simulink model "COMPONENT_MDL_Lag_QUAD_and_PEND_with_Ab"  (R2020b)
(part 12 of 12)

-m_pend.*(-THE_X_D+((Lz_pend.*THE_Psi_pend_D.*cos(THE_Theta_pend).*sin(THE_Psi_pend))./2.0+(Lz_pend.*THE_Theta_pend_D.*cos(THE_Psi_pend).*sin(THE_Theta_pend))./2.0).*(sin(THE_Phi).*sin(THE_Psi)+cos(THE_Phi).*cos(THE_Psi).*sin(THE_Theta))-(Tv_Z_pend+(Lz_pend.*cos(THE_Psi_pend).*cos(THE_Theta_pend))./2.0).*(THE_Phi_D.*cos(THE_Phi).*sin(THE_Psi)+THE_Psi_D.*cos(THE_Psi).*sin(THE_Phi)+THE_Theta_D.*cos(THE_Phi).*cos(THE_Psi).*cos(THE_Theta)-THE_Phi_D.*cos(THE_Psi).*sin(THE_Phi).*sin(THE_Theta)-THE_Psi_D.*cos(THE_Phi).*sin(THE_Psi).*sin(THE_Theta))+(Lz_pend.*(cos(THE_Phi_pend).*sin(THE_Psi_pend)-cos(THE_Psi_pend).*sin(THE_Phi_pend).*sin(THE_Theta_pend)).*(-THE_Phi_D.*cos(THE_Phi).*cos(THE_Psi)+THE_Psi_D.*sin(THE_Phi).*sin(THE_Psi)-THE_Phi_D.*sin(THE_Phi).*sin(THE_Psi).*sin(THE_Theta)+THE_Psi_D.*cos(THE_Phi).*cos(THE_Psi).*sin(THE_Theta)+THE_Theta_D.*cos(THE_Phi).*cos(THE_Theta).*sin(THE_Psi)))./2.0+(Lz_pend.*(cos(THE_Psi).*sin(THE_Phi)-cos(THE_Phi).*sin(THE_Psi).*sin(THE_Theta)).*(-THE_Psi_pend_D.*cos(THE_Phi_pend).*cos(THE_Psi_pend)+THE_Phi_pend_D.*sin(THE_Phi_pend).*sin(THE_Psi_pend)-THE_Psi_pend_D.*sin(THE_Phi_pend).*sin(THE_Psi_pend).*sin(THE_Theta_pend)+THE_Phi_pend_D.*cos(THE_Phi_pend).*cos(THE_Psi_pend).*sin(THE_Theta_pend)+THE_Theta_pend_D.*cos(THE_Psi_pend).*cos(THE_Theta_pend).*sin(THE_Phi_pend)))./2.0-(Lz_pend.*cos(THE_Phi).*cos(THE_Theta).*(THE_Phi_pend_D.*cos(THE_Phi_pend).*sin(THE_Psi_pend)+THE_Psi_pend_D.*cos(THE_Psi_pend).*sin(THE_Phi_pend)+THE_Theta_pend_D.*cos(THE_Phi_pend).*cos(THE_Psi_pend).*cos(THE_Theta_pend)-THE_Phi_pend_D.*cos(THE_Psi_pend).*sin(THE_Phi_pend).*sin(THE_Theta_pend)-THE_Psi_pend_D.*cos(THE_Phi_pend).*sin(THE_Psi_pend).*sin(THE_Theta_pend)))./2.0+(Lz_pend.*THE_Phi_D.*cos(THE_Theta).*sin(THE_Phi).*(sin(THE_Phi_pend).*sin(THE_Psi_pend)+cos(THE_Phi_pend).*cos(THE_Psi_pend).*sin(THE_Theta_pend)))./2.0+(Lz_pend.*THE_Theta_D.*cos(THE_Phi).*sin(THE_Theta).*(sin(THE_Phi_pend).*sin(THE_Psi_pend)+cos(THE_Phi_pend).*cos(THE_Psi_pend).*sin(THE_Theta_pend)))./2.0).*((Lz_pend.*(cos(THE_Phi_pend).*cos(THE_Psi_pend)+sin(THE_Phi_pend).*sin(THE_Psi_pend).*sin(THE_Theta_pend)).*(-THE_Phi_D.*cos(THE_Phi).*cos(THE_Psi)+THE_Psi_D.*sin(THE_Phi).*sin(THE_Psi)-THE_Phi_D.*sin(THE_Phi).*sin(THE_Psi).*sin(THE_Theta)+THE_Psi_D.*cos(THE_Phi).*cos(THE_Psi).*sin(THE_Theta)+THE_Theta_D.*cos(THE_Phi).*cos(THE_Theta).*sin(THE_Psi)))./4.0-(Lz_pend.*(cos(THE_Psi).*sin(THE_Phi)-cos(THE_Phi).*sin(THE_Psi).*sin(THE_Theta)).*(-THE_Phi_pend_D.*cos(THE_Psi_pend).*sin(THE_Phi_pend)-THE_Psi_pend_D.*cos(THE_Phi_pend).*sin(THE_Psi_pend)+THE_Phi_pend_D.*cos(THE_Phi_pend).*sin(THE_Psi_pend).*sin(THE_Theta_pend)+THE_Psi_pend_D.*cos(THE_Psi_pend).*sin(THE_Phi_pend).*sin(THE_Theta_pend)+THE_Theta_pend_D.*cos(THE_Theta_pend).*sin(THE_Phi_pend).*sin(THE_Psi_pend)))./4.0+(Lz_pend.*cos(THE_Theta_pend).*sin(THE_Psi_pend).*(THE_Phi_D.*cos(THE_Phi).*sin(THE_Psi)+THE_Psi_D.*cos(THE_Psi).*sin(THE_Phi)+THE_Theta_D.*cos(THE_Phi).*cos(THE_Psi).*cos(THE_Theta)-THE_Phi_D.*cos(THE_Psi).*sin(THE_Phi).*sin(THE_Theta)-THE_Psi_D.*cos(THE_Phi).*sin(THE_Psi).*sin(THE_Theta)))./4.0+(Lz_pend.*cos(THE_Phi).*cos(THE_Theta).*(-THE_Phi_pend_D.*cos(THE_Phi_pend).*cos(THE_Psi_pend)+THE_Psi_pend_D.*sin(THE_Phi_pend).*sin(THE_Psi_pend)-THE_Phi_pend_D.*sin(THE_Phi_pend).*sin(THE_Psi_pend).*sin(THE_Theta_pend)+THE_Psi_pend_D.*cos(THE_Phi_pend).*cos(THE_Psi_pend).*sin(THE_Theta_pend)+THE_Theta_pend_D.*cos(THE_Phi_pend).*cos(THE_Theta_pend).*sin(THE_Psi_pend)))./4.0+(Lz_pend.*THE_Psi_pend_D.*cos(THE_Psi_pend).*cos(THE_Theta_pend).*(sin(THE_Phi).*sin(THE_Psi)+cos(THE_Phi).*cos(THE_Psi).*sin(THE_Theta)))./4.0+(Lz_pend.*THE_Phi_D.*cos(THE_Theta).*sin(THE_Phi).*(cos(THE_Psi_pend).*sin(THE_Phi_pend)-cos(THE_Phi_pend).*sin(THE_Psi_pend).*sin(THE_Theta_pend)))./4.0+(Lz_pend.*THE_Theta_D.*cos(THE_Phi).*sin(THE_Theta).*(cos(THE_Psi_pend).*sin(THE_Phi_pend)-cos(THE_Phi_pend).*sin(THE_Psi_pend).*sin(THE_Theta_pend)))./4.0-(Lz_pend.*THE_Theta_pend_D.*sin(THE_Psi_pend).*sin(THE_Theta_pend).*(sin(THE_Phi).*sin(THE_Psi)+cos(THE_Phi).*cos(THE_Psi).*sin(THE_Theta)))./4.0)-m_pend.*(THE_X_D.*(-1.0./2.0)+(((Lz_pend.*THE_Psi_pend_D.*cos(THE_Theta_pend).*sin(THE_Psi_pend))./2.0+(Lz_pend.*THE_Theta_pend_D.*cos(THE_Psi_pend).*sin(THE_Theta_pend))./2.0).*(sin(THE_Phi).*sin(THE_Psi)+cos(THE_Phi).*cos(THE_Psi).*sin(THE_Theta)))./2.0-((Tv_Z_pend+(Lz_pend.*cos(THE_Psi_pend).*cos(THE_Theta_pend))./2.0).*(THE_Phi_D.*cos(THE_Phi).*sin(THE_Psi)+THE_Psi_D.*cos(THE_Psi).*sin(THE_Phi)+THE_Theta_D.*cos(THE_Phi).*cos(THE_Psi).*cos(THE_Theta)-THE_Phi_D.*cos(THE_Psi).*sin(THE_Phi).*sin(THE_Theta)-THE_Psi_D.*cos(THE_Phi).*sin(THE_Psi).*sin(THE_Theta)))./2.0+(Lz_pend.*(cos(THE_Phi_pend).*sin(THE_Psi_pend)-cos(THE_Psi_pend).*sin(THE_Phi_pend).*sin(THE_Theta_pend)).*(-THE_Phi_D.*cos(THE_Phi).*cos(THE_Psi)+THE_Psi_D.*sin(THE_Phi).*sin(THE_Psi)-THE_Phi_D.*sin(THE_Phi).*sin(THE_Psi).*sin(THE_Theta)+THE_Psi_D.*cos(THE_Phi).*cos(THE_Psi).*sin(THE_Theta)+THE_Theta_D.*cos(THE_Phi).*cos(THE_Theta).*sin(THE_Psi)))./4.0+(Lz_pend.*(cos(THE_Psi).*sin(THE_Phi)-cos(THE_Phi).*sin(THE_Psi).*sin(THE_Theta)).*(-THE_Psi_pend_D.*cos(THE_Phi_pend).*cos(THE_Psi_pend)+THE_Phi_pend_D.*sin(THE_Phi_pend).*sin(THE_Psi_pend)-THE_Psi_pend_D.*sin(THE_Phi_pend).*sin(THE_Psi_pend).*sin(THE_Theta_pend)+THE_Phi_pend_D.*cos(THE_Phi_pend).*cos(THE_Psi_pend).*sin(THE_Theta_pend)+THE_Theta_pend_D.*cos(THE_Psi_pend).*cos(THE_Theta_pend).*sin(THE_Phi_pend)))./4.0-(Lz_pend.*cos(THE_Phi).*cos(THE_Theta).*(THE_Phi_pend_D.*cos(THE_Phi_pend).*sin(THE_Psi_pend)+THE_Psi_pend_D.*cos(THE_Psi_pend).*sin(THE_Phi_pend)+THE_Theta_pend_D.*cos(THE_Phi_pend).*cos(THE_Psi_pend).*cos(THE_Theta_pend)-THE_Phi_pend_D.*cos(THE_Psi_pend).*sin(THE_Phi_pend).*sin(THE_Theta_pend)-THE_Psi_pend_D.*cos(THE_Phi_pend).*sin(THE_Psi_pend).*sin(THE_Theta_pend)))./4.0+(Lz_pend.*THE_Phi_D.*cos(THE_Theta).*sin(THE_Phi).*(sin(THE_Phi_pend).*sin(THE_Psi_pend)+cos(THE_Phi_pend).*cos(THE_Psi_pend).*sin(THE_Theta_pend)))./4.0+(Lz_pend.*THE_Theta_D.*cos(THE_Phi).*sin(THE_Theta).*(sin(THE_Phi_pend).*sin(THE_Psi_pend)+cos(THE_Phi_pend).*cos(THE_Psi_pend).*sin(THE_Theta_pend)))./4.0).*((Lz_pend.*(cos(THE_Phi_pend).*cos(THE_Psi_pend)+sin(THE_Phi_pend).*sin(THE_Psi_pend).*sin(THE_Theta_pend)).*(-THE_Phi_D.*cos(THE_Phi).*cos(THE_Psi)+THE_Psi_D.*sin(THE_Phi).*sin(THE_Psi)-THE_Phi_D.*sin(THE_Phi).*sin(THE_Psi).*sin(THE_Theta)+THE_Psi_D.*cos(THE_Phi).*cos(THE_Psi).*sin(THE_Theta)+THE_Theta_D.*cos(THE_Phi).*cos(THE_Theta).*sin(THE_Psi)))./2.0-(Lz_pend.*(cos(THE_Psi).*sin(THE_Phi)-cos(THE_Phi).*sin(THE_Psi).*sin(THE_Theta)).*(-THE_Phi_pend_D.*cos(THE_Psi_pend).*sin(THE_Phi_pend)-THE_Psi_pend_D.*cos(THE_Phi_pend).*sin(THE_Psi_pend)+THE_Phi_pend_D.*cos(THE_Phi_pend).*sin(THE_Psi_pend).*sin(THE_Theta_pend)+THE_Psi_pend_D.*cos(THE_Psi_pend).*sin(THE_Phi_pend).*sin(THE_Theta_pend)+THE_Theta_pend_D.*cos(THE_Theta_pend).*sin(THE_Phi_pend).*sin(THE_Psi_pend)))./2.0+(Lz_pend.*cos(THE_Theta_pend).*sin(THE_Psi_pend).*(THE_Phi_D.*cos(THE_Phi).*sin(THE_Psi)+THE_Psi_D.*cos(THE_Psi).*sin(THE_Phi)+THE_Theta_D.*cos(THE_Phi).*cos(THE_Psi).*cos(THE_Theta)-THE_Phi_D.*cos(THE_Psi).*sin(THE_Phi).*sin(THE_Theta)-THE_Psi_D.*cos(THE_Phi).*sin(THE_Psi).*sin(THE_Theta)))./2.0+(Lz_pend.*cos(THE_Phi).*cos(THE_Theta).*(-THE_Phi_pend_D.*cos(THE_Phi_pend).*cos(THE_Psi_pend)+THE_Psi_pend_D.*sin(THE_Phi_pend).*sin(THE_Psi_pend)-THE_Phi_pend_D.*sin(THE_Phi_pend).*sin(THE_Psi_pend).*sin(THE_Theta_pend)+THE_Psi_pend_D.*cos(THE_Phi_pend).*cos(THE_Psi_pend).*sin(THE_Theta_pend)+THE_Theta_pend_D.*cos(THE_Phi_pend).*cos(THE_Theta_pend).*sin(THE_Psi_pend)))./2.0+(Lz_pend.*THE_Psi_pend_D.*cos(THE_Psi_pend).*cos(THE_Theta_pend).*(sin(THE_Phi).*sin(THE_Psi)+cos(THE_Phi).*cos(THE_Psi).*sin(THE_Theta)))./2.0+(Lz_pend.*THE_Phi_D.*cos(THE_Theta).*sin(THE_Phi).*(cos(THE_Psi_pend).*sin(THE_Phi_pend)-cos(THE_Phi_pend).*sin(THE_Psi_pend).*sin(THE_Theta_pend)))./2.0+(Lz_pend.*THE_Theta_D.*cos(THE_Phi).*sin(THE_Theta).*(cos(THE_Psi_pend).*sin(THE_Phi_pend)-cos(THE_Phi_pend).*sin(THE_Psi_pend).*sin(THE_Theta_pend)))./2.0-(Lz_pend.*THE_Theta_pend_D.*sin(THE_Psi_pend).*sin(THE_Theta_pend).*(sin(THE_Phi).*sin(THE_Psi)+cos(THE_Phi).*cos(THE_Psi).*sin(THE_Theta)))./2.0)+m_pend.*((Lz_pend.*(cos(THE_Phi_pend).*cos(THE_Psi_pend)+sin(THE_Phi_pend).*sin(THE_Psi_pend).*sin(THE_Theta_pend)).*(-THE_Phi_D.*cos(THE_Psi).*sin(THE_Phi)-THE_Psi_D.*cos(THE_Phi).*sin(THE_Psi)+THE_Phi_D.*cos(THE_Phi).*sin(THE_Psi).*sin(THE_Theta)+THE_Psi_D.*cos(THE_Psi).*sin(THE_Phi).*sin(THE_Theta)+THE_Theta_D.*cos(THE_Theta).*sin(THE_Phi).*sin(THE_Psi)))./4.0+(Lz_pend.*(cos(THE_Phi).*cos(THE_Psi)+sin(THE_Phi).*sin(THE_Psi).*sin(THE_Theta)).*(-THE_Phi_pend_D.*cos(THE_Psi_pend).*sin(THE_Phi_pend)-THE_Psi_pend_D.*cos(THE_Phi_pend).*sin(THE_Psi_pend)+THE_Phi_pend_D.*cos(THE_Phi_pend).*sin(THE_Psi_pend).*sin(THE_Theta_pend)+THE_Psi_pend_D.*cos(THE_Psi_pend).*sin(THE_Phi_pend).*sin(THE_Theta_pend)+THE_Theta_pend_D.*cos(THE_Theta_pend).*sin(THE_Phi_pend).*sin(THE_Psi_pend)))./4.0+(Lz_pend.*cos(THE_Theta_pend).*sin(THE_Psi_pend).*(-THE_Psi_D.*cos(THE_Phi).*cos(THE_Psi)+THE_Phi_D.*sin(THE_Phi).*sin(THE_Psi)-THE_Psi_D.*sin(THE_Phi).*sin(THE_Psi).*sin(THE_Theta)+THE_Phi_D.*cos(THE_Phi).*cos(THE_Psi).*sin(THE_Theta)+THE_Theta_D.*cos(THE_Psi).*cos(THE_Theta).*sin(THE_Phi)))./4.0+(Lz_pend.*cos(THE_Theta).*sin(THE_Phi).*(-THE_Phi_pend_D.*cos(THE_Phi_pend).*cos(THE_Psi_pend)+THE_Psi_pend_D.*sin(THE_Phi_pend).*sin(THE_Psi_pend)-THE_Phi_pend_D.*sin(THE_Phi_pend).*sin(THE_Psi_pend).*sin(THE_Theta_pend)+THE_Psi_pend_D.*cos(THE_Phi_pend).*cos(THE_Psi_pend).*sin(THE_Theta_pend)+THE_Theta_pend_D.*cos(THE_Phi_pend).*cos(THE_Theta_pend).*sin(THE_Psi_pend)))./4.0-(Lz_pend.*THE_Psi_pend_D.*cos(THE_Psi_pend).*cos(THE_Theta_pend).*(cos(THE_Phi).*sin(THE_Psi)-cos(THE_Psi).*sin(THE_Phi).*sin(THE_Theta)))./4.0-(Lz_pend.*THE_Phi_D.*cos(THE_Phi).*cos(THE_Theta).*(cos(THE_Psi_pend).*sin(THE_Phi_pend)-cos(THE_Phi_pend).*sin(THE_Psi_pend).*sin(THE_Theta_pend)))./4.0+(Lz_pend.*THE_Theta_pend_D.*sin(THE_Psi_pend).*sin(THE_Theta_pend).*(cos(THE_Phi).*sin(THE_Psi)-cos(THE_Psi).*sin(THE_Phi).*sin(THE_Theta)))./4.0+(Lz_pend.*THE_Theta_D.*sin(THE_Phi).*sin(THE_Theta).*(cos(THE_Psi_pend).*sin(THE_Phi_pend)-cos(THE_Phi_pend).*sin(THE_Psi_pend).*sin(THE_Theta_pend)))./4.0).*(THE_Y_D+((Lz_pend.*THE_Psi_pend_D.*cos(THE_Theta_pend).*sin(THE_Psi_pend))./2.0+(Lz_pend.*THE_Theta_pend_D.*cos(THE_Psi_pend).*sin(THE_Theta_pend))./2.0).*(cos(THE_Phi).*sin(THE_Psi)-cos(THE_Psi).*sin(THE_Phi).*sin(THE_Theta))+(Tv_Z_pend+(Lz_pend.*cos(THE_Psi_pend).*cos(THE_Theta_pend))./2.0).*(-THE_Psi_D.*cos(THE_Phi).*cos(THE_Psi)+THE_Phi_D.*sin(THE_Phi).*sin(THE_Psi)-THE_Psi_D.*sin(THE_Phi).*sin(THE_Psi).*sin(THE_Theta)+THE_Phi_D.*cos(THE_Phi).*cos(THE_Psi).*sin(THE_Theta)+THE_Theta_D.*cos(THE_Psi).*cos(THE_Theta).*sin(THE_Phi))+(Lz_pend.*(cos(THE_Phi).*cos(THE_Psi)+sin(THE_Phi).*sin(THE_Psi).*sin(THE_Theta)).*(-THE_Psi_pend_D.*cos(THE_Phi_pend).*cos(THE_Psi_pend)+THE_Phi_pend_D.*sin(THE_Phi_pend).*sin(THE_Psi_pend)-THE_Psi_pend_D.*sin(THE_Phi_pend).*sin(THE_Psi_pend).*sin(THE_Theta_pend)+THE_Phi_pend_D.*cos(THE_Phi_pend).*cos(THE_Psi_pend).*sin(THE_Theta_pend)+THE_Theta_pend_D.*cos(THE_Psi_pend).*cos(THE_Theta_pend).*sin(THE_Phi_pend)))./2.0-(Lz_pend.*(cos(THE_Phi_pend).*sin(THE_Psi_pend)-cos(THE_Psi_pend).*sin(THE_Phi_pend).*sin(THE_Theta_pend)).*(-THE_Phi_D.*cos(THE_Psi).*sin(THE_Phi)-THE_Psi_D.*cos(THE_Phi).*sin(THE_Psi)+THE_Phi_D.*cos(THE_Phi).*sin(THE_Psi).*sin(THE_Theta)+THE_Psi_D.*cos(THE_Psi).*sin(THE_Phi).*sin(THE_Theta)+THE_Theta_D.*cos(THE_Theta).*sin(THE_Phi).*sin(THE_Psi)))./2.0+(Lz_pend.*cos(THE_Theta).*sin(THE_Phi).*(THE_Phi_pend_D.*cos(THE_Phi_pend).*sin(THE_Psi_pend)+THE_Psi_pend_D.*cos(THE_Psi_pend).*sin(THE_Phi_pend)+THE_Theta_pend_D.*cos(THE_Phi_pend).*cos(THE_Psi_pend).*cos(THE_Theta_pend)-THE_Phi_pend_D.*cos(THE_Psi_pend).*sin(THE_Phi_pend).*sin(THE_Theta_pend)-THE_Psi_pend_D.*cos(THE_Phi_pend).*sin(THE_Psi_pend).*sin(THE_Theta_pend)))./2.0+(Lz_pend.*THE_Phi_D.*cos(THE_Phi).*cos(THE_Theta).*(sin(THE_Phi_pend).*sin(THE_Psi_pend)+cos(THE_Phi_pend).*cos(THE_Psi_pend).*sin(THE_Theta_pend)))./2.0-(Lz_pend.*THE_Theta_D.*sin(THE_Phi).*sin(THE_Theta).*(sin(THE_Phi_pend).*sin(THE_Psi_pend)+cos(THE_Phi_pend).*cos(THE_Psi_pend).*sin(THE_Theta_pend)))./2.0)+m_pend.*(Lz_pend.*(cos(THE_Phi).*cos(THE_Psi)+sin(THE_Phi).*sin(THE_Psi).*sin(THE_Theta)).*(cos(THE_Phi_pend).*cos(THE_Psi_pend)+sin(THE_Phi_pend).*sin(THE_Psi_pend).*sin(THE_Theta_pend)).*(-1.0./4.0)+(Lz_pend.*cos(THE_Theta_pend).*sin(THE_Psi_pend).*(cos(THE_Phi).*sin(THE_Psi)-cos(THE_Psi).*sin(THE_Phi).*sin(THE_Theta)))./4.0+(Lz_pend.*cos(THE_Theta).*sin(THE_Phi).*(cos(THE_Psi_pend).*sin(THE_Phi_pend)-cos(THE_Phi_pend).*sin(THE_Psi_pend).*sin(THE_Theta_pend)))./4.0).*((Tv_Z_pend+(Lz_pend.*cos(THE_Psi_pend).*cos(THE_Theta_pend))./2.0).*(-THE_Phi_D.^2.*cos(THE_Phi).*sin(THE_Psi)-THE_Psi_D.^2.*cos(THE_Phi).*sin(THE_Psi)+THE_Phi_D.^2.*cos(THE_Psi).*sin(THE_Phi).*sin(THE_Theta)+THE_Psi_D.^2.*cos(THE_Psi).*sin(THE_Phi).*sin(THE_Theta)+THE_Theta_D.^2.*cos(THE_Psi).*sin(THE_Phi).*sin(THE_Theta)-THE_Phi_D.*THE_Psi_D.*cos(THE_Psi).*sin(THE_Phi).*2.0-THE_Phi_D.*THE_Theta_D.*cos(THE_Phi).*cos(THE_Psi).*cos(THE_Theta).*2.0+THE_Phi_D.*THE_Psi_D.*cos(THE_Phi).*sin(THE_Psi).*sin(THE_Theta).*2.0+THE_Psi_D.*THE_Theta_D.*cos(THE_Theta).*sin(THE_Phi).*sin(THE_Psi).*2.0)-(cos(THE_Phi).*sin(THE_Psi)-cos(THE_Psi).*sin(THE_Phi).*sin(THE_Theta)).*((Lz_pend.*THE_Psi_pend_D.^2.*cos(THE_Psi_pend).*cos(THE_Theta_pend))./2.0+(Lz_pend.*THE_Theta_pend_D.^2.*cos(THE_Psi_pend).*cos(THE_Theta_pend))./2.0-Lz_pend.*THE_Psi_pend_D.*THE_Theta_pend_D.*sin(THE_Psi_pend).*sin(THE_Theta_pend))+((Lz_pend.*THE_Psi_pend_D.*cos(THE_Theta_pend).*sin(THE_Psi_pend))./2.0+(Lz_pend.*THE_Theta_pend_D.*cos(THE_Psi_pend).*sin(THE_Theta_pend))./2.0).*(-THE_Psi_D.*cos(THE_Phi).*cos(THE_Psi)+THE_Phi_D.*sin(THE_Phi).*sin(THE_Psi)-THE_Psi_D.*sin(THE_Phi).*sin(THE_Psi).*sin(THE_Theta)+THE_Phi_D.*cos(THE_Phi).*cos(THE_Psi).*sin(THE_Theta)+THE_Theta_D.*cos(THE_Psi).*cos(THE_Theta).*sin(THE_Phi)).*2.0-Lz_pend.*(-THE_Psi_pend_D.*cos(THE_Phi_pend).*cos(THE_Psi_pend)+THE_Phi_pend_D.*sin(THE_Phi_pend).*sin(THE_Psi_pend)-THE_Psi_pend_D.*sin(THE_Phi_pend).*sin(THE_Psi_pend).*sin(THE_Theta_pend)+THE_Phi_pend_D.*cos(THE_Phi_pend).*cos(THE_Psi_pend).*sin(THE_Theta_pend)+THE_Theta_pend_D.*cos(THE_Psi_pend).*cos(THE_Theta_pend).*sin(THE_Phi_pend)).*(-THE_Phi_D.*cos(THE_Psi).*sin(THE_Phi)-THE_Psi_D.*cos(THE_Phi).*sin(THE_Psi)+THE_Phi_D.*cos(THE_Phi).*sin(THE_Psi).*sin(THE_Theta)+THE_Psi_D.*cos(THE_Psi).*sin(THE_Phi).*sin(THE_Theta)+THE_Theta_D.*cos(THE_Theta).*sin(THE_Phi).*sin(THE_Psi))+(Lz_pend.*(cos(THE_Phi).*cos(THE_Psi)+sin(THE_Phi).*sin(THE_Psi).*sin(THE_Theta)).*(-THE_Phi_pend_D.^2.*cos(THE_Phi_pend).*sin(THE_Psi_pend)-THE_Psi_pend_D.^2.*cos(THE_Phi_pend).*sin(THE_Psi_pend)+THE_Phi_pend_D.^2.*cos(THE_Psi_pend).*sin(THE_Phi_pend).*sin(THE_Theta_pend)+THE_Psi_pend_D.^2.*cos(THE_Psi_pend).*sin(THE_Phi_pend).*sin(THE_Theta_pend)+THE_Theta_pend_D.^2.*cos(THE_Psi_pend).*sin(THE_Phi_pend).*sin(THE_Theta_pend)-THE_Phi_pend_D.*THE_Psi_pend_D.*cos(THE_Psi_pend).*sin(THE_Phi_pend).*2.0-THE_Phi_pend_D.*THE_Theta_pend_D.*cos(THE_Phi_pend).*cos(THE_Psi_pend).*cos(THE_Theta_pend).*2.0+THE_Phi_pend_D.*THE_Psi_pend_D.*cos(THE_Phi_pend).*sin(THE_Psi_pend).*sin(THE_Theta_pend).*2.0+THE_Psi_pend_D.*THE_Theta_pend_D.*cos(THE_Theta_pend).*sin(THE_Phi_pend).*sin(THE_Psi_pend).*2.0))./2.0-(Lz_pend.*(cos(THE_Phi_pend).*sin(THE_Psi_pend)-cos(THE_Psi_pend).*sin(THE_Phi_pend).*sin(THE_Theta_pend)).*(THE_Phi_D.^2.*cos(THE_Phi).*cos(THE_Psi)+THE_Psi_D.^2.*cos(THE_Phi).*cos(THE_Psi)+THE_Phi_D.^2.*sin(THE_Phi).*sin(THE_Psi).*sin(THE_Theta)+THE_Psi_D.^2.*sin(THE_Phi).*sin(THE_Psi).*sin(THE_Theta)+THE_Theta_D.^2.*sin(THE_Phi).*sin(THE_Psi).*sin(THE_Theta)-THE_Phi_D.*THE_Psi_D.*sin(THE_Phi).*sin(THE_Psi).*2.0-THE_Phi_D.*THE_Psi_D.*cos(THE_Phi).*cos(THE_Psi).*sin(THE_Theta).*2.0-THE_Phi_D.*THE_Theta_D.*cos(THE_Phi).*cos(THE_Theta).*sin(THE_Psi).*2.0-THE_Psi_D.*THE_Theta_D.*cos(THE_Psi).*cos(THE_Theta).*sin(THE_Phi).*2.0))./2.0+(Lz_pend.*cos(THE_Theta).*sin(THE_Phi).*(THE_Phi_pend_D.^2.*sin(THE_Phi_pend).*sin(THE_Psi_pend)+THE_Psi_pend_D.^2.*sin(THE_Phi_pend).*sin(THE_Psi_pend)+THE_Phi_pend_D.^2.*cos(THE_Phi_pend).*cos(THE_Psi_pend).*sin(THE_Theta_pend)+THE_Psi_pend_D.^2.*cos(THE_Phi_pend).*cos(THE_Psi_pend).*sin(THE_Theta_pend)+THE_Theta_pend_D.^2.*cos(THE_Phi_pend).*cos(THE_Psi_pend).*sin(THE_Theta_pend)-THE_Phi_pend_D.*THE_Psi_pend_D.*cos(THE_Phi_pend).*cos(THE_Psi_pend).*2.0+THE_Phi_pend_D.*THE_Theta_pend_D.*cos(THE_Psi_pend).*cos(THE_Theta_pend).*sin(THE_Phi_pend).*2.0+THE_Psi_pend_D.*THE_Theta_pend_D.*cos(THE_Phi_pend).*cos(THE_Theta_pend).*sin(THE_Psi_pend).*2.0-THE_Phi_pend_D.*THE_Psi_pend_D.*sin(THE_Phi_pend).*sin(THE_Psi_pend).*sin(THE_Theta_pend).*2.0))./2.0-Lz_pend.*THE_Phi_D.*cos(THE_Phi).*cos(THE_Theta).*(THE_Phi_pend_D.*cos(THE_Phi_pend).*sin(THE_Psi_pend)+THE_Psi_pend_D.*cos(THE_Psi_pend).*sin(THE_Phi_pend)+THE_Theta_pend_D.*cos(THE_Phi_pend).*cos(THE_Psi_pend).*cos(THE_Theta_pend)-THE_Phi_pend_D.*cos(THE_Psi_pend).*sin(THE_Phi_pend).*sin(THE_Theta_pend)-THE_Psi_pend_D.*cos(THE_Phi_pend).*sin(THE_Psi_pend).*sin(THE_Theta_pend))+Lz_pend.*THE_Theta_D.*sin(THE_Phi).*sin(THE_Theta).*(THE_Phi_pend_D.*cos(THE_Phi_pend).*sin(THE_Psi_pend)+THE_Psi_pend_D.*cos(THE_Psi_pend).*sin(THE_Phi_pend)+THE_Theta_pend_D.*cos(THE_Phi_pend).*cos(THE_Psi_pend).*cos(THE_Theta_pend)-THE_Phi_pend_D.*cos(THE_Psi_pend).*sin(THE_Phi_pend).*sin(THE_Theta_pend)-THE_Psi_pend_D.*cos(THE_Phi_pend).*sin(THE_Psi_pend).*sin(THE_Theta_pend))+(Lz_pend.*THE_Phi_D.^2.*cos(THE_Theta).*sin(THE_Phi).*(sin(THE_Phi_pend).*sin(THE_Psi_pend)+cos(THE_Phi_pend).*cos(THE_Psi_pend).*sin(THE_Theta_pend)))./2.0+(Lz_pend.*THE_Theta_D.^2.*cos(THE_Theta).*sin(THE_Phi).*(sin(THE_Phi_pend).*sin(THE_Psi_pend)+cos(THE_Phi_pend).*cos(THE_Psi_pend).*sin(THE_Theta_pend)))./2.0+Lz_pend.*THE_Phi_D.*THE_Theta_D.*cos(THE_Phi).*sin(THE_Theta).*(sin(THE_Phi_pend).*sin(THE_Psi_pend)+cos(THE_Phi_pend).*cos(THE_Psi_pend).*sin(THE_Theta_pend)))+m_pend.*(Lz_pend.*(cos(THE_Phi).*cos(THE_Psi)+sin(THE_Phi).*sin(THE_Psi).*sin(THE_Theta)).*(cos(THE_Phi_pend).*cos(THE_Psi_pend)+sin(THE_Phi_pend).*sin(THE_Psi_pend).*sin(THE_Theta_pend)).*(-1.0./2.0)+(Lz_pend.*cos(THE_Theta_pend).*sin(THE_Psi_pend).*(cos(THE_Phi).*sin(THE_Psi)-cos(THE_Psi).*sin(THE_Phi).*sin(THE_Theta)))./2.0+(Lz_pend.*cos(THE_Theta).*sin(THE_Phi).*(cos(THE_Psi_pend).*sin(THE_Phi_pend)-cos(THE_Phi_pend).*sin(THE_Psi_pend).*sin(THE_Theta_pend)))./2.0).*(((Tv_Z_pend+(Lz_pend.*cos(THE_Psi_pend).*cos(THE_Theta_pend))./2.0).*(-THE_Phi_D.^2.*cos(THE_Phi).*sin(THE_Psi)-THE_Psi_D.^2.*cos(THE_Phi).*sin(THE_Psi)+THE_Phi_D.^2.*cos(THE_Psi).*sin(THE_Phi).*sin(THE_Theta)+THE_Psi_D.^2.*cos(THE_Psi).*sin(THE_Phi).*sin(THE_Theta)+THE_Theta_D.^2.*cos(THE_Psi).*sin(THE_Phi).*sin(THE_Theta)-THE_Phi_D.*THE_Psi_D.*cos(THE_Psi).*sin(THE_Phi).*2.0-THE_Phi_D.*THE_Theta_D.*cos(THE_Phi).*cos(THE_Psi).*cos(THE_Theta).*2.0+THE_Phi_D.*THE_Psi_D.*cos(THE_Phi).*sin(THE_Psi).*sin(THE_Theta).*2.0+THE_Psi_D.*THE_Theta_D.*cos(THE_Theta).*sin(THE_Phi).*sin(THE_Psi).*2.0))./2.0-((cos(THE_Phi).*sin(THE_Psi)-cos(THE_Psi).*sin(THE_Phi).*sin(THE_Theta)).*((Lz_pend.*THE_Psi_pend_D.^2.*cos(THE_Psi_pend).*cos(THE_Theta_pend))./2.0+(Lz_pend.*THE_Theta_pend_D.^2.*cos(THE_Psi_pend).*cos(THE_Theta_pend))./2.0-Lz_pend.*THE_Psi_pend_D.*THE_Theta_pend_D.*sin(THE_Psi_pend).*sin(THE_Theta_pend)))./2.0+((Lz_pend.*THE_Psi_pend_D.*cos(THE_Theta_pend).*sin(THE_Psi_pend))./2.0+(Lz_pend.*THE_Theta_pend_D.*cos(THE_Psi_pend).*sin(THE_Theta_pend))./2.0).*(-THE_Psi_D.*cos(THE_Phi).*cos(THE_Psi)+THE_Phi_D.*sin(THE_Phi).*sin(THE_Psi)-THE_Psi_D.*sin(THE_Phi).*sin(THE_Psi).*sin(THE_Theta)+THE_Phi_D.*cos(THE_Phi).*cos(THE_Psi).*sin(THE_Theta)+THE_Theta_D.*cos(THE_Psi).*cos(THE_Theta).*sin(THE_Phi))-(Lz_pend.*(-THE_Psi_pend_D.*cos(THE_Phi_pend).*cos(THE_Psi_pend)+THE_Phi_pend_D.*sin(THE_Phi_pend).*sin(THE_Psi_pend)-THE_Psi_pend_D.*sin(THE_Phi_pend).*sin(THE_Psi_pend).*sin(THE_Theta_pend)+THE_Phi_pend_D.*cos(THE_Phi_pend).*cos(THE_Psi_pend).*sin(THE_Theta_pend)+THE_Theta_pend_D.*cos(THE_Psi_pend).*cos(THE_Theta_pend).*sin(THE_Phi_pend)).*(-THE_Phi_D.*cos(THE_Psi).*sin(THE_Phi)-THE_Psi_D.*cos(THE_Phi).*sin(THE_Psi)+THE_Phi_D.*cos(THE_Phi).*sin(THE_Psi).*sin(THE_Theta)+THE_Psi_D.*cos(THE_Psi).*sin(THE_Phi).*sin(THE_Theta)+THE_Theta_D.*cos(THE_Theta).*sin(THE_Phi).*sin(THE_Psi)))./2.0+(Lz_pend.*(cos(THE_Phi).*cos(THE_Psi)+sin(THE_Phi).*sin(THE_Psi).*sin(THE_Theta)).*(-THE_Phi_pend_D.^2.*cos(THE_Phi_pend).*sin(THE_Psi_pend)-THE_Psi_pend_D.^2.*cos(THE_Phi_pend).*sin(THE_Psi_pend)+THE_Phi_pend_D.^2.*cos(THE_Psi_pend).*sin(THE_Phi_pend).*sin(THE_Theta_pend)+THE_Psi_pend_D.^2.*cos(THE_Psi_pend).*sin(THE_Phi_pend).*sin(THE_Theta_pend)+THE_Theta_pend_D.^2.*cos(THE_Psi_pend).*sin(THE_Phi_pend).*sin(THE_Theta_pend)-THE_Phi_pend_D.*THE_Psi_pend_D.*cos(THE_Psi_pend).*sin(THE_Phi_pend).*2.0-THE_Phi_pend_D.*THE_Theta_pend_D.*cos(THE_Phi_pend).*cos(THE_Psi_pend).*cos(THE_Theta_pend).*2.0+THE_Phi_pend_D.*THE_Psi_pend_D.*cos(THE_Phi_pend).*sin(THE_Psi_pend).*sin(THE_Theta_pend).*2.0+THE_Psi_pend_D.*THE_Theta_pend_D.*cos(THE_Theta_pend).*sin(THE_Phi_pend).*sin(THE_Psi_pend).*2.0))./4.0-(Lz_pend.*(cos(THE_Phi_pend).*sin(THE_Psi_pend)-cos(THE_Psi_pend).*sin(THE_Phi_pend).*sin(THE_Theta_pend)).*(THE_Phi_D.^2.*cos(THE_Phi).*cos(THE_Psi)+THE_Psi_D.^2.*cos(THE_Phi).*cos(THE_Psi)+THE_Phi_D.^2.*sin(THE_Phi).*sin(THE_Psi).*sin(THE_Theta)+THE_Psi_D.^2.*sin(THE_Phi).*sin(THE_Psi).*sin(THE_Theta)+THE_Theta_D.^2.*sin(THE_Phi).*sin(THE_Psi).*sin(THE_Theta)-THE_Phi_D.*THE_Psi_D.*sin(THE_Phi).*sin(THE_Psi).*2.0-THE_Phi_D.*THE_Psi_D.*cos(THE_Phi).*cos(THE_Psi).*sin(THE_Theta).*2.0-THE_Phi_D.*THE_Theta_D.*cos(THE_Phi).*cos(THE_Theta).*sin(THE_Psi).*2.0-THE_Psi_D.*THE_Theta_D.*cos(THE_Psi).*cos(THE_Theta).*sin(THE_Phi).*2.0))./4.0+(Lz_pend.*cos(THE_Theta).*sin(THE_Phi).*(THE_Phi_pend_D.^2.*sin(THE_Phi_pend).*sin(THE_Psi_pend)+THE_Psi_pend_D.^2.*sin(THE_Phi_pend).*sin(THE_Psi_pend)+THE_Phi_pend_D.^2.*cos(THE_Phi_pend).*cos(THE_Psi_pend).*sin(THE_Theta_pend)+THE_Psi_pend_D.^2.*cos(THE_Phi_pend).*cos(THE_Psi_pend).*sin(THE_Theta_pend)+THE_Theta_pend_D.^2.*cos(THE_Phi_pend).*cos(THE_Psi_pend).*sin(THE_Theta_pend)-THE_Phi_pend_D.*THE_Psi_pend_D.*cos(THE_Phi_pend).*cos(THE_Psi_pend).*2.0+THE_Phi_pend_D.*THE_Theta_pend_D.*cos(THE_Psi_pend).*cos(THE_Theta_pend).*sin(THE_Phi_pend).*2.0+THE_Psi_pend_D.*THE_Theta_pend_D.*cos(THE_Phi_pend).*cos(THE_Theta_pend).*sin(THE_Psi_pend).*2.0-THE_Phi_pend_D.*THE_Psi_pend_D.*sin(THE_Phi_pend).*sin(THE_Psi_pend).*sin(THE_Theta_pend).*2.0))./4.0-(Lz_pend.*THE_Phi_D.*cos(THE_Phi).*cos(THE_Theta).*(THE_Phi_pend_D.*cos(THE_Phi_pend).*sin(THE_Psi_pend)+THE_Psi_pend_D.*cos(THE_Psi_pend).*sin(THE_Phi_pend)+THE_Theta_pend_D.*cos(THE_Phi_pend).*cos(THE_Psi_pend).*cos(THE_Theta_pend)-THE_Phi_pend_D.*cos(THE_Psi_pend).*sin(THE_Phi_pend).*sin(THE_Theta_pend)-THE_Psi_pend_D.*cos(THE_Phi_pend).*sin(THE_Psi_pend).*sin(THE_Theta_pend)))./2.0+(Lz_pend.*THE_Theta_D.*sin(THE_Phi).*sin(THE_Theta).*(THE_Phi_pend_D.*cos(THE_Phi_pend).*sin(THE_Psi_pend)+THE_Psi_pend_D.*cos(THE_Psi_pend).*sin(THE_Phi_pend)+THE_Theta_pend_D.*cos(THE_Phi_pend).*cos(THE_Psi_pend).*cos(THE_Theta_pend)-THE_Phi_pend_D.*cos(THE_Psi_pend).*sin(THE_Phi_pend).*sin(THE_Theta_pend)-THE_Psi_pend_D.*cos(THE_Phi_pend).*sin(THE_Psi_pend).*sin(THE_Theta_pend)))./2.0+(Lz_pend.*THE_Phi_D.^2.*cos(THE_Theta).*sin(THE_Phi).*(sin(THE_Phi_pend).*sin(THE_Psi_pend)+cos(THE_Phi_pend).*cos(THE_Psi_pend).*sin(THE_Theta_pend)))./4.0+(Lz_pend.*THE_Theta_D.^2.*cos(THE_Theta).*sin(THE_Phi).*(sin(THE_Phi_pend).*sin(THE_Psi_pend)+cos(THE_Phi_pend).*cos(THE_Psi_pend).*sin(THE_Theta_pend)))./4.0+(Lz_pend.*THE_Phi_D.*THE_Theta_D.*cos(THE_Phi).*sin(THE_Theta).*(sin(THE_Phi_pend).*sin(THE_Psi_pend)+cos(THE_Phi_pend).*cos(THE_Psi_pend).*sin(THE_Theta_pend)))./2.0)-m_pend.*((Lz_pend.*sin(THE_Theta).*(-THE_Phi_pend_D.*cos(THE_Phi_pend).*cos(THE_Psi_pend)+THE_Psi_pend_D.*sin(THE_Phi_pend).*sin(THE_Psi_pend)-THE_Phi_pend_D.*sin(THE_Phi_pend).*sin(THE_Psi_pend).*sin(THE_Theta_pend)+THE_Psi_pend_D.*cos(THE_Phi_pend).*cos(THE_Psi_pend).*sin(THE_Theta_pend)+THE_Theta_pend_D.*cos(THE_Phi_pend).*cos(THE_Theta_pend).*sin(THE_Psi_pend)))./4.0-(cos(THE_Psi).*cos(THE_Theta).*((Lz_pend.*THE_Psi_pend_D.*cos(THE_Psi_pend).*cos(THE_Theta_pend))./2.0-(Lz_pend.*THE_Theta_pend_D.*sin(THE_Psi_pend).*sin(THE_Theta_pend))./2.0))./2.0-(Lz_pend.*THE_Theta_D.*cos(THE_Theta).*(cos(THE_Psi_pend).*sin(THE_Phi_pend)-cos(THE_Phi_pend).*sin(THE_Psi_pend).*sin(THE_Theta_pend)))./4.0-(Lz_pend.*cos(THE_Theta).*sin(THE_Psi).*(-THE_Phi_pend_D.*cos(THE_Psi_pend).*sin(THE_Phi_pend)-THE_Psi_pend_D.*cos(THE_Phi_pend).*sin(THE_Psi_pend)+THE_Phi_pend_D.*cos(THE_Phi_pend).*sin(THE_Psi_pend).*sin(THE_Theta_pend)+THE_Psi_pend_D.*cos(THE_Psi_pend).*sin(THE_Phi_pend).*sin(THE_Theta_pend)+THE_Theta_pend_D.*cos(THE_Theta_pend).*sin(THE_Phi_pend).*sin(THE_Psi_pend)))./4.0-(Lz_pend.*THE_Psi_D.*cos(THE_Psi).*cos(THE_Theta).*(cos(THE_Phi_pend).*cos(THE_Psi_pend)+sin(THE_Phi_pend).*sin(THE_Psi_pend).*sin(THE_Theta_pend)))./4.0+(Lz_pend.*THE_Theta_D.*sin(THE_Psi).*sin(THE_Theta).*(cos(THE_Phi_pend).*cos(THE_Psi_pend)+sin(THE_Phi_pend).*sin(THE_Psi_pend).*sin(THE_Theta_pend)))./4.0+(Lz_pend.*THE_Psi_D.*cos(THE_Theta).*cos(THE_Theta_pend).*sin(THE_Psi).*sin(THE_Psi_pend))./4.0+(Lz_pend.*THE_Theta_D.*cos(THE_Psi).*cos(THE_Theta_pend).*sin(THE_Theta).*sin(THE_Psi_pend))./4.0).*(-THE_Z_D+(Lz_pend.*sin(THE_Theta).*(THE_Phi_pend_D.*cos(THE_Phi_pend).*sin(THE_Psi_pend)+THE_Psi_pend_D.*cos(THE_Psi_pend).*sin(THE_Phi_pend)+THE_Theta_pend_D.*cos(THE_Phi_pend).*cos(THE_Psi_pend).*cos(THE_Theta_pend)-THE_Phi_pend_D.*cos(THE_Psi_pend).*sin(THE_Phi_pend).*sin(THE_Theta_pend)-THE_Psi_pend_D.*cos(THE_Phi_pend).*sin(THE_Psi_pend).*sin(THE_Theta_pend)))./2.0+cos(THE_Psi).*cos(THE_Theta).*((Lz_pend.*THE_Psi_pend_D.*cos(THE_Theta_pend).*sin(THE_Psi_pend))./2.0+(Lz_pend.*THE_Theta_pend_D.*cos(THE_Psi_pend).*sin(THE_Theta_pend))./2.0)+THE_Psi_D.*cos(THE_Theta).*sin(THE_Psi).*(Tv_Z_pend+(Lz_pend.*cos(THE_Psi_pend).*cos(THE_Theta_pend))./2.0)+THE_Theta_D.*cos(THE_Psi).*sin(THE_Theta).*(Tv_Z_pend+(Lz_pend.*cos(THE_Psi_pend).*cos(THE_Theta_pend))./2.0)+(Lz_pend.*THE_Theta_D.*cos(THE_Theta).*(sin(THE_Phi_pend).*sin(THE_Psi_pend)+cos(THE_Phi_pend).*cos(THE_Psi_pend).*sin(THE_Theta_pend)))./2.0-(Lz_pend.*cos(THE_Theta).*sin(THE_Psi).*(-THE_Psi_pend_D.*cos(THE_Phi_pend).*cos(THE_Psi_pend)+THE_Phi_pend_D.*sin(THE_Phi_pend).*sin(THE_Psi_pend)-THE_Psi_pend_D.*sin(THE_Phi_pend).*sin(THE_Psi_pend).*sin(THE_Theta_pend)+THE_Phi_pend_D.*cos(THE_Phi_pend).*cos(THE_Psi_pend).*sin(THE_Theta_pend)+THE_Theta_pend_D.*cos(THE_Psi_pend).*cos(THE_Theta_pend).*sin(THE_Phi_pend)))./2.0+(Lz_pend.*THE_Psi_D.*cos(THE_Psi).*cos(THE_Theta).*(cos(THE_Phi_pend).*sin(THE_Psi_pend)-cos(THE_Psi_pend).*sin(THE_Phi_pend).*sin(THE_Theta_pend)))./2.0-(Lz_pend.*THE_Theta_D.*sin(THE_Psi).*sin(THE_Theta).*(cos(THE_Phi_pend).*sin(THE_Psi_pend)-cos(THE_Psi_pend).*sin(THE_Phi_pend).*sin(THE_Theta_pend)))./2.0)-m_pend.*((Lz_pend.*sin(THE_Theta).*(-THE_Phi_pend_D.*cos(THE_Phi_pend).*cos(THE_Psi_pend)+THE_Psi_pend_D.*sin(THE_Phi_pend).*sin(THE_Psi_pend)-THE_Phi_pend_D.*sin(THE_Phi_pend).*sin(THE_Psi_pend).*sin(THE_Theta_pend)+THE_Psi_pend_D.*cos(THE_Phi_pend).*cos(THE_Psi_pend).*sin(THE_Theta_pend)+THE_Theta_pend_D.*cos(THE_Phi_pend).*cos(THE_Theta_pend).*sin(THE_Psi_pend)))./2.0-cos(THE_Psi).*cos(THE_Theta).*((Lz_pend.*THE_Psi_pend_D.*cos(THE_Psi_pend).*cos(THE_Theta_pend))./2.0-(Lz_pend.*THE_Theta_pend_D.*sin(THE_Psi_pend).*sin(THE_Theta_pend))./2.0)-(Lz_pend.*THE_Theta_D.*cos(THE_Theta).*(cos(THE_Psi_pend).*sin(THE_Phi_pend)-cos(THE_Phi_pend).*sin(THE_Psi_pend).*sin(THE_Theta_pend)))./2.0-(Lz_pend.*cos(THE_Theta).*sin(THE_Psi).*(-THE_Phi_pend_D.*cos(THE_Psi_pend).*sin(THE_Phi_pend)-THE_Psi_pend_D.*cos(THE_Phi_pend).*sin(THE_Psi_pend)+THE_Phi_pend_D.*cos(THE_Phi_pend).*sin(THE_Psi_pend).*sin(THE_Theta_pend)+THE_Psi_pend_D.*cos(THE_Psi_pend).*sin(THE_Phi_pend).*sin(THE_Theta_pend)+THE_Theta_pend_D.*cos(THE_Theta_pend).*sin(THE_Phi_pend).*sin(THE_Psi_pend)))./2.0-(Lz_pend.*THE_Psi_D.*cos(THE_Psi).*cos(THE_Theta).*(cos(THE_Phi_pend).*cos(THE_Psi_pend)+sin(THE_Phi_pend).*sin(THE_Psi_pend).*sin(THE_Theta_pend)))./2.0+(Lz_pend.*THE_Theta_D.*sin(THE_Psi).*sin(THE_Theta).*(cos(THE_Phi_pend).*cos(THE_Psi_pend)+sin(THE_Phi_pend).*sin(THE_Psi_pend).*sin(THE_Theta_pend)))./2.0+(Lz_pend.*THE_Psi_D.*cos(THE_Theta).*cos(THE_Theta_pend).*sin(THE_Psi).*sin(THE_Psi_pend))./2.0+(Lz_pend.*THE_Theta_D.*cos(THE_Psi).*cos(THE_Theta_pend).*sin(THE_Theta).*sin(THE_Psi_pend))./2.0).*(THE_Z_D.*(-1.0./2.0)+(Lz_pend.*sin(THE_Theta).*(THE_Phi_pend_D.*cos(THE_Phi_pend).*sin(THE_Psi_pend)+THE_Psi_pend_D.*cos(THE_Psi_pend).*sin(THE_Phi_pend)+THE_Theta_pend_D.*cos(THE_Phi_pend).*cos(THE_Psi_pend).*cos(THE_Theta_pend)-THE_Phi_pend_D.*cos(THE_Psi_pend).*sin(THE_Phi_pend).*sin(THE_Theta_pend)-THE_Psi_pend_D.*cos(THE_Phi_pend).*sin(THE_Psi_pend).*sin(THE_Theta_pend)))./4.0+(cos(THE_Psi).*cos(THE_Theta).*((Lz_pend.*THE_Psi_pend_D.*cos(THE_Theta_pend).*sin(THE_Psi_pend))./2.0+(Lz_pend.*THE_Theta_pend_D.*cos(THE_Psi_pend).*sin(THE_Theta_pend))./2.0))./2.0+(THE_Psi_D.*cos(THE_Theta).*sin(THE_Psi).*(Tv_Z_pend+(Lz_pend.*cos(THE_Psi_pend).*cos(THE_Theta_pend))./2.0))./2.0+(THE_Theta_D.*cos(THE_Psi).*sin(THE_Theta).*(Tv_Z_pend+(Lz_pend.*cos(THE_Psi_pend).*cos(THE_Theta_pend))./2.0))./2.0+(Lz_pend.*THE_Theta_D.*cos(THE_Theta).*(sin(THE_Phi_pend).*sin(THE_Psi_pend)+cos(THE_Phi_pend).*cos(THE_Psi_pend).*sin(THE_Theta_pend)))./4.0-(Lz_pend.*cos(THE_Theta).*sin(THE_Psi).*(-THE_Psi_pend_D.*cos(THE_Phi_pend).*cos(THE_Psi_pend)+THE_Phi_pend_D.*sin(THE_Phi_pend).*sin(THE_Psi_pend)-THE_Psi_pend_D.*sin(THE_Phi_pend).*sin(THE_Psi_pend).*sin(THE_Theta_pend)+THE_Phi_pend_D.*cos(THE_Phi_pend).*cos(THE_Psi_pend).*sin(THE_Theta_pend)+THE_Theta_pend_D.*cos(THE_Psi_pend).*cos(THE_Theta_pend).*sin(THE_Phi_pend)))./4.0+(Lz_pend.*THE_Psi_D.*cos(THE_Psi).*cos(THE_Theta).*(cos(THE_Phi_pend).*sin(THE_Psi_pend)-cos(THE_Psi_pend).*sin(THE_Phi_pend).*sin(THE_Theta_pend)))./4.0-(Lz_pend.*THE_Theta_D.*sin(THE_Psi).*sin(THE_Theta).*(cos(THE_Phi_pend).*sin(THE_Psi_pend)-cos(THE_Psi_pend).*sin(THE_Phi_pend).*sin(THE_Theta_pend)))./4.0)-m_pend.*(-((Lz_pend.*THE_Psi_pend_D.*cos(THE_Psi_pend).*cos(THE_Theta_pend))./2.0-(Lz_pend.*THE_Theta_pend_D.*sin(THE_Psi_pend).*sin(THE_Theta_pend))./2.0).*(cos(THE_Phi).*sin(THE_Psi)-cos(THE_Psi).*sin(THE_Phi).*sin(THE_Theta))+(Lz_pend.*(cos(THE_Phi_pend).*cos(THE_Psi_pend)+sin(THE_Phi_pend).*sin(THE_Psi_pend).*sin(THE_Theta_pend)).*(-THE_Phi_D.*cos(THE_Psi).*sin(THE_Phi)-THE_Psi_D.*cos(THE_Phi).*sin(THE_Psi)+THE_Phi_D.*cos(THE_Phi).*sin(THE_Psi).*sin(THE_Theta)+THE_Psi_D.*cos(THE_Psi).*sin(THE_Phi).*sin(THE_Theta)+THE_Theta_D.*cos(THE_Theta).*sin(THE_Phi).*sin(THE_Psi)))./2.0+(Lz_pend.*(cos(THE_Phi).*cos(THE_Psi)+sin(THE_Phi).*sin(THE_Psi).*sin(THE_Theta)).*(-THE_Phi_pend_D.*cos(THE_Psi_pend).*sin(THE_Phi_pend)-THE_Psi_pend_D.*cos(THE_Phi_pend).*sin(THE_Psi_pend)+THE_Phi_pend_D.*cos(THE_Phi_pend).*sin(THE_Psi_pend).*sin(THE_Theta_pend)+THE_Psi_pend_D.*cos(THE_Psi_pend).*sin(THE_Phi_pend).*sin(THE_Theta_pend)+THE_Theta_pend_D.*cos(THE_Theta_pend).*sin(THE_Phi_pend).*sin(THE_Psi_pend)))./2.0+(Lz_pend.*cos(THE_Theta_pend).*sin(THE_Psi_pend).*(-THE_Psi_D.*cos(THE_Phi).*cos(THE_Psi)+THE_Phi_D.*sin(THE_Phi).*sin(THE_Psi)-THE_Psi_D.*sin(THE_Phi).*sin(THE_Psi).*sin(THE_Theta)+THE_Phi_D.*cos(THE_Phi).*cos(THE_Psi).*sin(THE_Theta)+THE_Theta_D.*cos(THE_Psi).*cos(THE_Theta).*sin(THE_Phi)))./2.0+(Lz_pend.*cos(THE_Theta).*sin(THE_Phi).*(-THE_Phi_pend_D.*cos(THE_Phi_pend).*cos(THE_Psi_pend)+THE_Psi_pend_D.*sin(THE_Phi_pend).*sin(THE_Psi_pend)-THE_Phi_pend_D.*sin(THE_Phi_pend).*sin(THE_Psi_pend).*sin(THE_Theta_pend)+THE_Psi_pend_D.*cos(THE_Phi_pend).*cos(THE_Psi_pend).*sin(THE_Theta_pend)+THE_Theta_pend_D.*cos(THE_Phi_pend).*cos(THE_Theta_pend).*sin(THE_Psi_pend)))./2.0-(Lz_pend.*THE_Phi_D.*cos(THE_Phi).*cos(THE_Theta).*(cos(THE_Psi_pend).*sin(THE_Phi_pend)-cos(THE_Phi_pend).*sin(THE_Psi_pend).*sin(THE_Theta_pend)))./2.0+(Lz_pend.*THE_Theta_D.*sin(THE_Phi).*sin(THE_Theta).*(cos(THE_Psi_pend).*sin(THE_Phi_pend)-cos(THE_Phi_pend).*sin(THE_Psi_pend).*sin(THE_Theta_pend)))./2.0).*(THE_Y_D./2.0+(((Lz_pend.*THE_Psi_pend_D.*cos(THE_Theta_pend).*sin(THE_Psi_pend))./2.0+(Lz_pend.*THE_Theta_pend_D.*cos(THE_Psi_pend).*sin(THE_Theta_pend))./2.0).*(cos(THE_Phi).*sin(THE_Psi)-cos(THE_Psi).*sin(THE_Phi).*sin(THE_Theta)))./2.0+((Tv_Z_pend+(Lz_pend.*cos(THE_Psi_pend).*cos(THE_Theta_pend))./2.0).*(-THE_Psi_D.*cos(THE_Phi).*cos(THE_Psi)+THE_Phi_D.*sin(THE_Phi).*sin(THE_Psi)-THE_Psi_D.*sin(THE_Phi).*sin(THE_Psi).*sin(THE_Theta)+THE_Phi_D.*cos(THE_Phi).*cos(THE_Psi).*sin(THE_Theta)+THE_Theta_D.*cos(THE_Psi).*cos(THE_Theta).*sin(THE_Phi)))./2.0+(Lz_pend.*(cos(THE_Phi).*cos(THE_Psi)+sin(THE_Phi).*sin(THE_Psi).*sin(THE_Theta)).*(-THE_Psi_pend_D.*cos(THE_Phi_pend).*cos(THE_Psi_pend)+THE_Phi_pend_D.*sin(THE_Phi_pend).*sin(THE_Psi_pend)-THE_Psi_pend_D.*sin(THE_Phi_pend).*sin(THE_Psi_pend).*sin(THE_Theta_pend)+THE_Phi_pend_D.*cos(THE_Phi_pend).*cos(THE_Psi_pend).*sin(THE_Theta_pend)+THE_Theta_pend_D.*cos(THE_Psi_pend).*cos(THE_Theta_pend).*sin(THE_Phi_pend)))./4.0-(Lz_pend.*(cos(THE_Phi_pend).*sin(THE_Psi_pend)-cos(THE_Psi_pend).*sin(THE_Phi_pend).*sin(THE_Theta_pend)).*(-THE_Phi_D.*cos(THE_Psi).*sin(THE_Phi)-THE_Psi_D.*cos(THE_Phi).*sin(THE_Psi)+THE_Phi_D.*cos(THE_Phi).*sin(THE_Psi).*sin(THE_Theta)+THE_Psi_D.*cos(THE_Psi).*sin(THE_Phi).*sin(THE_Theta)+THE_Theta_D.*cos(THE_Theta).*sin(THE_Phi).*sin(THE_Psi)))./4.0+(Lz_pend.*cos(THE_Theta).*sin(THE_Phi).*(THE_Phi_pend_D.*cos(THE_Phi_pend).*sin(THE_Psi_pend)+THE_Psi_pend_D.*cos(THE_Psi_pend).*sin(THE_Phi_pend)+THE_Theta_pend_D.*cos(THE_Phi_pend).*cos(THE_Psi_pend).*cos(THE_Theta_pend)-THE_Phi_pend_D.*cos(THE_Psi_pend).*sin(THE_Phi_pend).*sin(THE_Theta_pend)-THE_Psi_pend_D.*cos(THE_Phi_pend).*sin(THE_Psi_pend).*sin(THE_Theta_pend)))./4.0+(Lz_pend.*THE_Phi_D.*cos(THE_Phi).*cos(THE_Theta).*(sin(THE_Phi_pend).*sin(THE_Psi_pend)+cos(THE_Phi_pend).*cos(THE_Psi_pend).*sin(THE_Theta_pend)))./4.0-(Lz_pend.*THE_Theta_D.*sin(THE_Phi).*sin(THE_Theta).*(sin(THE_Phi_pend).*sin(THE_Psi_pend)+cos(THE_Phi_pend).*cos(THE_Psi_pend).*sin(THE_Theta_pend)))./4.0)+m_pend.*((Lz_pend.*(cos(THE_Phi_pend).*cos(THE_Psi_pend)+sin(THE_Phi_pend).*sin(THE_Psi_pend).*sin(THE_Theta_pend)).*(-THE_Phi_D.*cos(THE_Psi).*sin(THE_Phi)-THE_Psi_D.*cos(THE_Phi).*sin(THE_Psi)+THE_Phi_D.*cos(THE_Phi).*sin(THE_Psi).*sin(THE_Theta)+THE_Psi_D.*cos(THE_Psi).*sin(THE_Phi).*sin(THE_Theta)+THE_Theta_D.*cos(THE_Theta).*sin(THE_Phi).*sin(THE_Psi)))./2.0+(Lz_pend.*(cos(THE_Phi).*cos(THE_Psi)+sin(THE_Phi).*sin(THE_Psi).*sin(THE_Theta)).*(-THE_Phi_pend_D.*cos(THE_Psi_pend).*sin(THE_Phi_pend)-THE_Psi_pend_D.*cos(THE_Phi_pend).*sin(THE_Psi_pend)+THE_Phi_pend_D.*cos(THE_Phi_pend).*sin(THE_Psi_pend).*sin(THE_Theta_pend)+THE_Psi_pend_D.*cos(THE_Psi_pend).*sin(THE_Phi_pend).*sin(THE_Theta_pend)+THE_Theta_pend_D.*cos(THE_Theta_pend).*sin(THE_Phi_pend).*sin(THE_Psi_pend)))./2.0+(Lz_pend.*cos(THE_Theta_pend).*sin(THE_Psi_pend).*(-THE_Psi_D.*cos(THE_Phi).*cos(THE_Psi)+THE_Phi_D.*sin(THE_Phi).*sin(THE_Psi)-THE_Psi_D.*sin(THE_Phi).*sin(THE_Psi).*sin(THE_Theta)+THE_Phi_D.*cos(THE_Phi).*cos(THE_Psi).*sin(THE_Theta)+THE_Theta_D.*cos(THE_Psi).*cos(THE_Theta).*sin(THE_Phi)))./2.0+(Lz_pend.*cos(THE_Theta).*sin(THE_Phi).*(-THE_Phi_pend_D.*cos(THE_Phi_pend).*cos(THE_Psi_pend)+THE_Psi_pend_D.*sin(THE_Phi_pend).*sin(THE_Psi_pend)-THE_Phi_pend_D.*sin(THE_Phi_pend).*sin(THE_Psi_pend).*sin(THE_Theta_pend)+THE_Psi_pend_D.*cos(THE_Phi_pend).*cos(THE_Psi_pend).*sin(THE_Theta_pend)+THE_Theta_pend_D.*cos(THE_Phi_pend).*cos(THE_Theta_pend).*sin(THE_Psi_pend)))./2.0-(Lz_pend.*THE_Psi_pend_D.*cos(THE_Psi_pend).*cos(THE_Theta_pend).*(cos(THE_Phi).*sin(THE_Psi)-cos(THE_Psi).*sin(THE_Phi).*sin(THE_Theta)))./2.0-(Lz_pend.*THE_Phi_D.*cos(THE_Phi).*cos(THE_Theta).*(cos(THE_Psi_pend).*sin(THE_Phi_pend)-cos(THE_Phi_pend).*sin(THE_Psi_pend).*sin(THE_Theta_pend)))./2.0+(Lz_pend.*THE_Theta_pend_D.*sin(THE_Psi_pend).*sin(THE_Theta_pend).*(cos(THE_Phi).*sin(THE_Psi)-cos(THE_Psi).*sin(THE_Phi).*sin(THE_Theta)))./2.0+(Lz_pend.*THE_Theta_D.*sin(THE_Phi).*sin(THE_Theta).*(cos(THE_Psi_pend).*sin(THE_Phi_pend)-cos(THE_Phi_pend).*sin(THE_Psi_pend).*sin(THE_Theta_pend)))./2.0).*(THE_Y_D./2.0+(((Lz_pend.*THE_Psi_pend_D.*cos(THE_Theta_pend).*sin(THE_Psi_pend))./2.0+(Lz_pend.*THE_Theta_pend_D.*cos(THE_Psi_pend).*sin(THE_Theta_pend))./2.0).*(cos(THE_Phi).*sin(THE_Psi)-cos(THE_Psi).*sin(THE_Phi).*sin(THE_Theta)))./2.0+((Tv_Z_pend+(Lz_pend.*cos(THE_Psi_pend).*cos(THE_Theta_pend))./2.0).*(-THE_Psi_D.*cos(THE_Phi).*cos(THE_Psi)+THE_Phi_D.*sin(THE_Phi).*sin(THE_Psi)-THE_Psi_D.*sin(THE_Phi).*sin(THE_Psi).*sin(THE_Theta)+THE_Phi_D.*cos(THE_Phi).*cos(THE_Psi).*sin(THE_Theta)+THE_Theta_D.*cos(THE_Psi).*cos(THE_Theta).*sin(THE_Phi)))./2.0+(Lz_pend.*(cos(THE_Phi).*cos(THE_Psi)+sin(THE_Phi).*sin(THE_Psi).*sin(THE_Theta)).*(-THE_Psi_pend_D.*cos(THE_Phi_pend).*cos(THE_Psi_pend)+THE_Phi_pend_D.*sin(THE_Phi_pend).*sin(THE_Psi_pend)-THE_Psi_pend_D.*sin(THE_Phi_pend).*sin(THE_Psi_pend).*sin(THE_Theta_pend)+THE_Phi_pend_D.*cos(THE_Phi_pend).*cos(THE_Psi_pend).*sin(THE_Theta_pend)+THE_Theta_pend_D.*cos(THE_Psi_pend).*cos(THE_Theta_pend).*sin(THE_Phi_pend)))./4.0-(Lz_pend.*(cos(THE_Phi_pend).*sin(THE_Psi_pend)-cos(THE_Psi_pend).*sin(THE_Phi_pend).*sin(THE_Theta_pend)).*(-THE_Phi_D.*cos(THE_Psi).*sin(THE_Phi)-THE_Psi_D.*cos(THE_Phi).*sin(THE_Psi)+THE_Phi_D.*cos(THE_Phi).*sin(THE_Psi).*sin(THE_Theta)+THE_Psi_D.*cos(THE_Psi).*sin(THE_Phi).*sin(THE_Theta)+THE_Theta_D.*cos(THE_Theta).*sin(THE_Phi).*sin(THE_Psi)))./4.0+(Lz_pend.*cos(THE_Theta).*sin(THE_Phi).*(THE_Phi_pend_D.*cos(THE_Phi_pend).*sin(THE_Psi_pend)+THE_Psi_pend_D.*cos(THE_Psi_pend).*sin(THE_Phi_pend)+THE_Theta_pend_D.*cos(THE_Phi_pend).*cos(THE_Psi_pend).*cos(THE_Theta_pend)-THE_Phi_pend_D.*cos(THE_Psi_pend).*sin(THE_Phi_pend).*sin(THE_Theta_pend)-THE_Psi_pend_D.*cos(THE_Phi_pend).*sin(THE_Psi_pend).*sin(THE_Theta_pend)))./4.0+(Lz_pend.*THE_Phi_D.*cos(THE_Phi).*cos(THE_Theta).*(sin(THE_Phi_pend).*sin(THE_Psi_pend)+cos(THE_Phi_pend).*cos(THE_Psi_pend).*sin(THE_Theta_pend)))./4.0-(Lz_pend.*THE_Theta_D.*sin(THE_Phi).*sin(THE_Theta).*(sin(THE_Phi_pend).*sin(THE_Psi_pend)+cos(THE_Phi_pend).*cos(THE_Psi_pend).*sin(THE_Theta_pend)))./4.0)+(m_pend.*(Ly_pend.^2./1.2e+1+Lz_pend.^2./1.2e+1).*(-sin(THE_Theta_pend).*(THE_Psi_D.*THE_Theta_D.*cos(THE_Psi)+THE_Phi_D.*THE_Psi_D.*cos(THE_Theta).*sin(THE_Psi)+THE_Phi_D.*THE_Theta_D.*cos(THE_Psi).*sin(THE_Theta))+cos(THE_Theta_pend).*sin(THE_Phi_pend).*(THE_Psi_D.*THE_Theta_D.*sin(THE_Psi)-THE_Phi_D.*THE_Psi_D.*cos(THE_Psi).*cos(THE_Theta)+THE_Phi_D.*THE_Theta_D.*sin(THE_Psi).*sin(THE_Theta))-THE_Theta_pend_D.*cos(THE_Theta_pend).*(THE_Theta_D.*sin(THE_Psi)-THE_Phi_D.*cos(THE_Psi).*cos(THE_Theta))+THE_Phi_pend_D.*THE_Theta_pend_D.*cos(THE_Theta_pend)-THE_Phi_pend_D.*cos(THE_Phi_pend).*cos(THE_Theta_pend).*(THE_Theta_D.*cos(THE_Psi)+THE_Phi_D.*cos(THE_Theta).*sin(THE_Psi))+THE_Theta_pend_D.*sin(THE_Phi_pend).*sin(THE_Theta_pend).*(THE_Theta_D.*cos(THE_Psi)+THE_Phi_D.*cos(THE_Theta).*sin(THE_Psi))+THE_Phi_pend_D.*cos(THE_Theta_pend).*sin(THE_Phi_pend).*(THE_Psi_D-THE_Phi_D.*sin(THE_Theta))+THE_Theta_pend_D.*cos(THE_Phi_pend).*sin(THE_Theta_pend).*(THE_Psi_D-THE_Phi_D.*sin(THE_Theta))+THE_Phi_D.*THE_Theta_D.*cos(THE_Theta).*cos(THE_Phi_pend).*cos(THE_Theta_pend)))./2.0+m_pend.*(Ly_pend.^2./1.2e+1+Lz_pend.^2./1.2e+1).*(sin(THE_Theta_pend).*(THE_Psi_D.*THE_Theta_D.*cos(THE_Psi)+THE_Phi_D.*THE_Psi_D.*cos(THE_Theta).*sin(THE_Psi)+THE_Phi_D.*THE_Theta_D.*cos(THE_Psi).*sin(THE_Theta)).*(-1.0./2.0)+(cos(THE_Theta_pend).*sin(THE_Phi_pend).*(THE_Psi_D.*THE_Theta_D.*sin(THE_Psi)-THE_Phi_D.*THE_Psi_D.*cos(THE_Psi).*cos(THE_Theta)+THE_Phi_D.*THE_Theta_D.*sin(THE_Psi).*sin(THE_Theta)))./2.0-(THE_Theta_pend_D.*cos(THE_Theta_pend).*(THE_Theta_D.*sin(THE_Psi)-THE_Phi_D.*cos(THE_Psi).*cos(THE_Theta)))./2.0+(THE_Phi_pend_D.*THE_Theta_pend_D.*cos(THE_Theta_pend))./2.0-(THE_Phi_pend_D.*cos(THE_Phi_pend).*cos(THE_Theta_pend).*(THE_Theta_D.*cos(THE_Psi)+THE_Phi_D.*cos(THE_Theta).*sin(THE_Psi)))./2.0+(THE_Theta_pend_D.*sin(THE_Phi_pend).*sin(THE_Theta_pend).*(THE_Theta_D.*cos(THE_Psi)+THE_Phi_D.*cos(THE_Theta).*sin(THE_Psi)))./2.0+(THE_Phi_pend_D.*cos(THE_Theta_pend).*sin(THE_Phi_pend).*(THE_Psi_D-THE_Phi_D.*sin(THE_Theta)))./2.0+(THE_Theta_pend_D.*cos(THE_Phi_pend).*sin(THE_Theta_pend).*(THE_Psi_D-THE_Phi_D.*sin(THE_Theta)))./2.0+(THE_Phi_D.*THE_Theta_D.*cos(THE_Theta).*cos(THE_Phi_pend).*cos(THE_Theta_pend))./2.0)+g.*m_pend.*((Lz_pend.*sin(THE_Theta).*(cos(THE_Psi_pend).*sin(THE_Phi_pend)-cos(THE_Phi_pend).*sin(THE_Psi_pend).*sin(THE_Theta_pend)))./2.0+(Lz_pend.*cos(THE_Theta).*sin(THE_Psi).*(cos(THE_Phi_pend).*cos(THE_Psi_pend)+sin(THE_Phi_pend).*sin(THE_Psi_pend).*sin(THE_Theta_pend)))./2.0+(Lz_pend.*cos(THE_Psi).*cos(THE_Theta).*cos(THE_Theta_pend).*sin(THE_Psi_pend))./2.0)+m_pend.*((Lz_pend.*sin(THE_Theta).*(cos(THE_Psi_pend).*sin(THE_Phi_pend)-cos(THE_Phi_pend).*sin(THE_Psi_pend).*sin(THE_Theta_pend)))./4.0+(Lz_pend.*cos(THE_Theta).*sin(THE_Psi).*(cos(THE_Phi_pend).*cos(THE_Psi_pend)+sin(THE_Phi_pend).*sin(THE_Psi_pend).*sin(THE_Theta_pend)))./4.0+(Lz_pend.*cos(THE_Psi).*cos(THE_Theta).*cos(THE_Theta_pend).*sin(THE_Psi_pend))./4.0).*((Lz_pend.*sin(THE_Theta).*(THE_Phi_pend_D.^2.*sin(THE_Phi_pend).*sin(THE_Psi_pend)+THE_Psi_pend_D.^2.*sin(THE_Phi_pend).*sin(THE_Psi_pend)+THE_Phi_pend_D.^2.*cos(THE_Phi_pend).*cos(THE_Psi_pend).*sin(THE_Theta_pend)+THE_Psi_pend_D.^2.*cos(THE_Phi_pend).*cos(THE_Psi_pend).*sin(THE_Theta_pend)+THE_Theta_pend_D.^2.*cos(THE_Phi_pend).*cos(THE_Psi_pend).*sin(THE_Theta_pend)-THE_Phi_pend_D.*THE_Psi_pend_D.*cos(THE_Phi_pend).*cos(THE_Psi_pend).*2.0+THE_Phi_pend_D.*THE_Theta_pend_D.*cos(THE_Psi_pend).*cos(THE_Theta_pend).*sin(THE_Phi_pend).*2.0+THE_Psi_pend_D.*THE_Theta_pend_D.*cos(THE_Phi_pend).*cos(THE_Theta_pend).*sin(THE_Psi_pend).*2.0-THE_Phi_pend_D.*THE_Psi_pend_D.*sin(THE_Phi_pend).*sin(THE_Psi_pend).*sin(THE_Theta_pend).*2.0))./2.0-cos(THE_Psi).*cos(THE_Theta).*((Lz_pend.*THE_Psi_pend_D.^2.*cos(THE_Psi_pend).*cos(THE_Theta_pend))./2.0+(Lz_pend.*THE_Theta_pend_D.^2.*cos(THE_Psi_pend).*cos(THE_Theta_pend))./2.0-Lz_pend.*THE_Psi_pend_D.*THE_Theta_pend_D.*sin(THE_Psi_pend).*sin(THE_Theta_pend))+(Lz_pend.*THE_Theta_D.^2.*sin(THE_Theta).*(sin(THE_Phi_pend).*sin(THE_Psi_pend)+cos(THE_Phi_pend).*cos(THE_Psi_pend).*sin(THE_Theta_pend)))./2.0-(Lz_pend.*cos(THE_Theta).*sin(THE_Psi).*(-THE_Phi_pend_D.^2.*cos(THE_Phi_pend).*sin(THE_Psi_pend)-THE_Psi_pend_D.^2.*cos(THE_Phi_pend).*sin(THE_Psi_pend)+THE_Phi_pend_D.^2.*cos(THE_Psi_pend).*sin(THE_Phi_pend).*sin(THE_Theta_pend)+THE_Psi_pend_D.^2.*cos(THE_Psi_pend).*sin(THE_Phi_pend).*sin(THE_Theta_pend)+THE_Theta_pend_D.^2.*cos(THE_Psi_pend).*sin(THE_Phi_pend).*sin(THE_Theta_pend)-THE_Phi_pend_D.*THE_Psi_pend_D.*cos(THE_Psi_pend).*sin(THE_Phi_pend).*2.0-THE_Phi_pend_D.*THE_Theta_pend_D.*cos(THE_Phi_pend).*cos(THE_Psi_pend).*cos(THE_Theta_pend).*2.0+THE_Phi_pend_D.*THE_Psi_pend_D.*cos(THE_Phi_pend).*sin(THE_Psi_pend).*sin(THE_Theta_pend).*2.0+THE_Psi_pend_D.*THE_Theta_pend_D.*cos(THE_Theta_pend).*sin(THE_Phi_pend).*sin(THE_Psi_pend).*2.0))./2.0-Lz_pend.*THE_Theta_D.*cos(THE_Theta).*(THE_Phi_pend_D.*cos(THE_Phi_pend).*sin(THE_Psi_pend)+THE_Psi_pend_D.*cos(THE_Psi_pend).*sin(THE_Phi_pend)+THE_Theta_pend_D.*cos(THE_Phi_pend).*cos(THE_Psi_pend).*cos(THE_Theta_pend)-THE_Phi_pend_D.*cos(THE_Psi_pend).*sin(THE_Phi_pend).*sin(THE_Theta_pend)-THE_Psi_pend_D.*cos(THE_Phi_pend).*sin(THE_Psi_pend).*sin(THE_Theta_pend))-THE_Psi_D.^2.*cos(THE_Psi).*cos(THE_Theta).*(Tv_Z_pend+(Lz_pend.*cos(THE_Psi_pend).*cos(THE_Theta_pend))./2.0)-THE_Theta_D.^2.*cos(THE_Psi).*cos(THE_Theta).*(Tv_Z_pend+(Lz_pend.*cos(THE_Psi_pend).*cos(THE_Theta_pend))./2.0)+THE_Psi_D.*cos(THE_Theta).*sin(THE_Psi).*((Lz_pend.*THE_Psi_pend_D.*cos(THE_Theta_pend).*sin(THE_Psi_pend))./2.0+(Lz_pend.*THE_Theta_pend_D.*cos(THE_Psi_pend).*sin(THE_Theta_pend))./2.0).*2.0+THE_Theta_D.*cos(THE_Psi).*sin(THE_Theta).*((Lz_pend.*THE_Psi_pend_D.*cos(THE_Theta_pend).*sin(THE_Psi_pend))./2.0+(Lz_pend.*THE_Theta_pend_D.*cos(THE_Psi_pend).*sin(THE_Theta_pend))./2.0).*2.0+Lz_pend.*THE_Psi_D.*cos(THE_Psi).*cos(THE_Theta).*(-THE_Psi_pend_D.*cos(THE_Phi_pend).*cos(THE_Psi_pend)+THE_Phi_pend_D.*sin(THE_Phi_pend).*sin(THE_Psi_pend)-THE_Psi_pend_D.*sin(THE_Phi_pend).*sin(THE_Psi_pend).*sin(THE_Theta_pend)+THE_Phi_pend_D.*cos(THE_Phi_pend).*cos(THE_Psi_pend).*sin(THE_Theta_pend)+THE_Theta_pend_D.*cos(THE_Psi_pend).*cos(THE_Theta_pend).*sin(THE_Phi_pend))-Lz_pend.*THE_Theta_D.*sin(THE_Psi).*sin(THE_Theta).*(-THE_Psi_pend_D.*cos(THE_Phi_pend).*cos(THE_Psi_pend)+THE_Phi_pend_D.*sin(THE_Phi_pend).*sin(THE_Psi_pend)-THE_Psi_pend_D.*sin(THE_Phi_pend).*sin(THE_Psi_pend).*sin(THE_Theta_pend)+THE_Phi_pend_D.*cos(THE_Phi_pend).*cos(THE_Psi_pend).*sin(THE_Theta_pend)+THE_Theta_pend_D.*cos(THE_Psi_pend).*cos(THE_Theta_pend).*sin(THE_Phi_pend))+THE_Psi_D.*THE_Theta_D.*sin(THE_Psi).*sin(THE_Theta).*(Tv_Z_pend+(Lz_pend.*cos(THE_Psi_pend).*cos(THE_Theta_pend))./2.0).*2.0+(Lz_pend.*THE_Psi_D.^2.*cos(THE_Theta).*sin(THE_Psi).*(cos(THE_Phi_pend).*sin(THE_Psi_pend)-cos(THE_Psi_pend).*sin(THE_Phi_pend).*sin(THE_Theta_pend)))./2.0+(Lz_pend.*THE_Theta_D.^2.*cos(THE_Theta).*sin(THE_Psi).*(cos(THE_Phi_pend).*sin(THE_Psi_pend)-cos(THE_Psi_pend).*sin(THE_Phi_pend).*sin(THE_Theta_pend)))./2.0+Lz_pend.*THE_Psi_D.*THE_Theta_D.*cos(THE_Psi).*sin(THE_Theta).*(cos(THE_Phi_pend).*sin(THE_Psi_pend)-cos(THE_Psi_pend).*sin(THE_Phi_pend).*sin(THE_Theta_pend)))+m_pend.*((Lz_pend.*sin(THE_Theta).*(cos(THE_Psi_pend).*sin(THE_Phi_pend)-cos(THE_Phi_pend).*sin(THE_Psi_pend).*sin(THE_Theta_pend)))./2.0+(Lz_pend.*cos(THE_Theta).*sin(THE_Psi).*(cos(THE_Phi_pend).*cos(THE_Psi_pend)+sin(THE_Phi_pend).*sin(THE_Psi_pend).*sin(THE_Theta_pend)))./2.0+(Lz_pend.*cos(THE_Psi).*cos(THE_Theta).*cos(THE_Theta_pend).*sin(THE_Psi_pend))./2.0).*((Lz_pend.*sin(THE_Theta).*(THE_Phi_pend_D.^2.*sin(THE_Phi_pend).*sin(THE_Psi_pend)+THE_Psi_pend_D.^2.*sin(THE_Phi_pend).*sin(THE_Psi_pend)+THE_Phi_pend_D.^2.*cos(THE_Phi_pend).*cos(THE_Psi_pend).*sin(THE_Theta_pend)+THE_Psi_pend_D.^2.*cos(THE_Phi_pend).*cos(THE_Psi_pend).*sin(THE_Theta_pend)+THE_Theta_pend_D.^2.*cos(THE_Phi_pend).*cos(THE_Psi_pend).*sin(THE_Theta_pend)-THE_Phi_pend_D.*THE_Psi_pend_D.*cos(THE_Phi_pend).*cos(THE_Psi_pend).*2.0+THE_Phi_pend_D.*THE_Theta_pend_D.*cos(THE_Psi_pend).*cos(THE_Theta_pend).*sin(THE_Phi_pend).*2.0+THE_Psi_pend_D.*THE_Theta_pend_D.*cos(THE_Phi_pend).*cos(THE_Theta_pend).*sin(THE_Psi_pend).*2.0-THE_Phi_pend_D.*THE_Psi_pend_D.*sin(THE_Phi_pend).*sin(THE_Psi_pend).*sin(THE_Theta_pend).*2.0))./4.0-(cos(THE_Psi).*cos(THE_Theta).*((Lz_pend.*THE_Psi_pend_D.^2.*cos(THE_Psi_pend).*cos(THE_Theta_pend))./2.0+(Lz_pend.*THE_Theta_pend_D.^2.*cos(THE_Psi_pend).*cos(THE_Theta_pend))./2.0-Lz_pend.*THE_Psi_pend_D.*THE_Theta_pend_D.*sin(THE_Psi_pend).*sin(THE_Theta_pend)))./2.0+(Lz_pend.*THE_Theta_D.^2.*sin(THE_Theta).*(sin(THE_Phi_pend).*sin(THE_Psi_pend)+cos(THE_Phi_pend).*cos(THE_Psi_pend).*sin(THE_Theta_pend)))./4.0-(Lz_pend.*cos(THE_Theta).*sin(THE_Psi).*(-THE_Phi_pend_D.^2.*cos(THE_Phi_pend).*sin(THE_Psi_pend)-THE_Psi_pend_D.^2.*cos(THE_Phi_pend).*sin(THE_Psi_pend)+THE_Phi_pend_D.^2.*cos(THE_Psi_pend).*sin(THE_Phi_pend).*sin(THE_Theta_pend)+THE_Psi_pend_D.^2.*cos(THE_Psi_pend).*sin(THE_Phi_pend).*sin(THE_Theta_pend)+THE_Theta_pend_D.^2.*cos(THE_Psi_pend).*sin(THE_Phi_pend).*sin(THE_Theta_pend)-THE_Phi_pend_D.*THE_Psi_pend_D.*cos(THE_Psi_pend).*sin(THE_Phi_pend).*2.0-THE_Phi_pend_D.*THE_Theta_pend_D.*cos(THE_Phi_pend).*cos(THE_Psi_pend).*cos(THE_Theta_pend).*2.0+THE_Phi_pend_D.*THE_Psi_pend_D.*cos(THE_Phi_pend).*sin(THE_Psi_pend).*sin(THE_Theta_pend).*2.0+THE_Psi_pend_D.*THE_Theta_pend_D.*cos(THE_Theta_pend).*sin(THE_Phi_pend).*sin(THE_Psi_pend).*2.0))./4.0-(Lz_pend.*THE_Theta_D.*cos(THE_Theta).*(THE_Phi_pend_D.*cos(THE_Phi_pend).*sin(THE_Psi_pend)+THE_Psi_pend_D.*cos(THE_Psi_pend).*sin(THE_Phi_pend)+THE_Theta_pend_D.*cos(THE_Phi_pend).*cos(THE_Psi_pend).*cos(THE_Theta_pend)-THE_Phi_pend_D.*cos(THE_Psi_pend).*sin(THE_Phi_pend).*sin(THE_Theta_pend)-THE_Psi_pend_D.*cos(THE_Phi_pend).*sin(THE_Psi_pend).*sin(THE_Theta_pend)))./2.0-(THE_Psi_D.^2.*cos(THE_Psi).*cos(THE_Theta).*(Tv_Z_pend+(Lz_pend.*cos(THE_Psi_pend).*cos(THE_Theta_pend))./2.0))./2.0-(THE_Theta_D.^2.*cos(THE_Psi).*cos(THE_Theta).*(Tv_Z_pend+(Lz_pend.*cos(THE_Psi_pend).*cos(THE_Theta_pend))./2.0))./2.0+THE_Psi_D.*cos(THE_Theta).*sin(THE_Psi).*((Lz_pend.*THE_Psi_pend_D.*cos(THE_Theta_pend).*sin(THE_Psi_pend))./2.0+(Lz_pend.*THE_Theta_pend_D.*cos(THE_Psi_pend).*sin(THE_Theta_pend))./2.0)+THE_Theta_D.*cos(THE_Psi).*sin(THE_Theta).*((Lz_pend.*THE_Psi_pend_D.*cos(THE_Theta_pend).*sin(THE_Psi_pend))./2.0+(Lz_pend.*THE_Theta_pend_D.*cos(THE_Psi_pend).*sin(THE_Theta_pend))./2.0)+(Lz_pend.*THE_Psi_D.*cos(THE_Psi).*cos(THE_Theta).*(-THE_Psi_pend_D.*cos(THE_Phi_pend).*cos(THE_Psi_pend)+THE_Phi_pend_D.*sin(THE_Phi_pend).*sin(THE_Psi_pend)-THE_Psi_pend_D.*sin(THE_Phi_pend).*sin(THE_Psi_pend).*sin(THE_Theta_pend)+THE_Phi_pend_D.*cos(THE_Phi_pend).*cos(THE_Psi_pend).*sin(THE_Theta_pend)+THE_Theta_pend_D.*cos(THE_Psi_pend).*cos(THE_Theta_pend).*sin(THE_Phi_pend)))./2.0-(Lz_pend.*THE_Theta_D.*sin(THE_Psi).*sin(THE_Theta).*(-THE_Psi_pend_D.*cos(THE_Phi_pend).*cos(THE_Psi_pend)+THE_Phi_pend_D.*sin(THE_Phi_pend).*sin(THE_Psi_pend)-THE_Psi_pend_D.*sin(THE_Phi_pend).*sin(THE_Psi_pend).*sin(THE_Theta_pend)+THE_Phi_pend_D.*cos(THE_Phi_pend).*cos(THE_Psi_pend).*sin(THE_Theta_pend)+THE_Theta_pend_D.*cos(THE_Psi_pend).*cos(THE_Theta_pend).*sin(THE_Phi_pend)))./2.0+THE_Psi_D.*THE_Theta_D.*sin(THE_Psi).*sin(THE_Theta).*(Tv_Z_pend+(Lz_pend.*cos(THE_Psi_pend).*cos(THE_Theta_pend))./2.0)+(Lz_pend.*THE_Psi_D.^2.*cos(THE_Theta).*sin(THE_Psi).*(cos(THE_Phi_pend).*sin(THE_Psi_pend)-cos(THE_Psi_pend).*sin(THE_Phi_pend).*sin(THE_Theta_pend)))./4.0+(Lz_pend.*THE_Theta_D.^2.*cos(THE_Theta).*sin(THE_Psi).*(cos(THE_Phi_pend).*sin(THE_Psi_pend)-cos(THE_Psi_pend).*sin(THE_Phi_pend).*sin(THE_Theta_pend)))./4.0+(Lz_pend.*THE_Psi_D.*THE_Theta_D.*cos(THE_Psi).*sin(THE_Theta).*(cos(THE_Phi_pend).*sin(THE_Psi_pend)-cos(THE_Psi_pend).*sin(THE_Phi_pend).*sin(THE_Theta_pend)))./2.0)+m_pend.*((Lz_pend.*(cos(THE_Psi).*sin(THE_Phi)-cos(THE_Phi).*sin(THE_Psi).*sin(THE_Theta)).*(cos(THE_Phi_pend).*cos(THE_Psi_pend)+sin(THE_Phi_pend).*sin(THE_Psi_pend).*sin(THE_Theta_pend)))./4.0+(Lz_pend.*cos(THE_Phi).*cos(THE_Theta).*(cos(THE_Psi_pend).*sin(THE_Phi_pend)-cos(THE_Phi_pend).*sin(THE_Psi_pend).*sin(THE_Theta_pend)))./4.0-(Lz_pend.*cos(THE_Theta_pend).*sin(THE_Psi_pend).*(sin(THE_Phi).*sin(THE_Psi)+cos(THE_Phi).*cos(THE_Psi).*sin(THE_Theta)))./4.0).*((Tv_Z_pend+(Lz_pend.*cos(THE_Psi_pend).*cos(THE_Theta_pend))./2.0).*(THE_Phi_D.^2.*sin(THE_Phi).*sin(THE_Psi)+THE_Psi_D.^2.*sin(THE_Phi).*sin(THE_Psi)+THE_Phi_D.^2.*cos(THE_Phi).*cos(THE_Psi).*sin(THE_Theta)+THE_Psi_D.^2.*cos(THE_Phi).*cos(THE_Psi).*sin(THE_Theta)+THE_Theta_D.^2.*cos(THE_Phi).*cos(THE_Psi).*sin(THE_Theta)-THE_Phi_D.*THE_Psi_D.*cos(THE_Phi).*cos(THE_Psi).*2.0+THE_Phi_D.*THE_Theta_D.*cos(THE_Psi).*cos(THE_Theta).*sin(THE_Phi).*2.0+THE_Psi_D.*THE_Theta_D.*cos(THE_Phi).*cos(THE_Theta).*sin(THE_Psi).*2.0-THE_Phi_D.*THE_Psi_D.*sin(THE_Phi).*sin(THE_Psi).*sin(THE_Theta).*2.0)+(sin(THE_Phi).*sin(THE_Psi)+cos(THE_Phi).*cos(THE_Psi).*sin(THE_Theta)).*((Lz_pend.*THE_Psi_pend_D.^2.*cos(THE_Psi_pend).*cos(THE_Theta_pend))./2.0+(Lz_pend.*THE_Theta_pend_D.^2.*cos(THE_Psi_pend).*cos(THE_Theta_pend))./2.0-Lz_pend.*THE_Psi_pend_D.*THE_Theta_pend_D.*sin(THE_Psi_pend).*sin(THE_Theta_pend))+((Lz_pend.*THE_Psi_pend_D.*cos(THE_Theta_pend).*sin(THE_Psi_pend))./2.0+(Lz_pend.*THE_Theta_pend_D.*cos(THE_Psi_pend).*sin(THE_Theta_pend))./2.0).*(THE_Phi_D.*cos(THE_Phi).*sin(THE_Psi)+THE_Psi_D.*cos(THE_Psi).*sin(THE_Phi)+THE_Theta_D.*cos(THE_Phi).*cos(THE_Psi).*cos(THE_Theta)-THE_Phi_D.*cos(THE_Psi).*sin(THE_Phi).*sin(THE_Theta)-THE_Psi_D.*cos(THE_Phi).*sin(THE_Psi).*sin(THE_Theta)).*2.0-(Lz_pend.*(cos(THE_Phi_pend).*sin(THE_Psi_pend)-cos(THE_Psi_pend).*sin(THE_Phi_pend).*sin(THE_Theta_pend)).*(-THE_Phi_D.^2.*cos(THE_Psi).*sin(THE_Phi)-THE_Psi_D.^2.*cos(THE_Psi).*sin(THE_Phi)+THE_Phi_D.^2.*cos(THE_Phi).*sin(THE_Psi).*sin(THE_Theta)+THE_Psi_D.^2.*cos(THE_Phi).*sin(THE_Psi).*sin(THE_Theta)+THE_Theta_D.^2.*cos(THE_Phi).*sin(THE_Psi).*sin(THE_Theta)-THE_Phi_D.*THE_Psi_D.*cos(THE_Phi).*sin(THE_Psi).*2.0-THE_Psi_D.*THE_Theta_D.*cos(THE_Phi).*cos(THE_Psi).*cos(THE_Theta).*2.0+THE_Phi_D.*THE_Psi_D.*cos(THE_Psi).*sin(THE_Phi).*sin(THE_Theta).*2.0+THE_Phi_D.*THE_Theta_D.*cos(THE_Theta).*sin(THE_Phi).*sin(THE_Psi).*2.0))./2.0-(Lz_pend.*(cos(THE_Psi).*sin(THE_Phi)-cos(THE_Phi).*sin(THE_Psi).*sin(THE_Theta)).*(-THE_Phi_pend_D.^2.*cos(THE_Phi_pend).*sin(THE_Psi_pend)-THE_Psi_pend_D.^2.*cos(THE_Phi_pend).*sin(THE_Psi_pend)+THE_Phi_pend_D.^2.*cos(THE_Psi_pend).*sin(THE_Phi_pend).*sin(THE_Theta_pend)+THE_Psi_pend_D.^2.*cos(THE_Psi_pend).*sin(THE_Phi_pend).*sin(THE_Theta_pend)+THE_Theta_pend_D.^2.*cos(THE_Psi_pend).*sin(THE_Phi_pend).*sin(THE_Theta_pend)-THE_Phi_pend_D.*THE_Psi_pend_D.*cos(THE_Psi_pend).*sin(THE_Phi_pend).*2.0-THE_Phi_pend_D.*THE_Theta_pend_D.*cos(THE_Phi_pend).*cos(THE_Psi_pend).*cos(THE_Theta_pend).*2.0+THE_Phi_pend_D.*THE_Psi_pend_D.*cos(THE_Phi_pend).*sin(THE_Psi_pend).*sin(THE_Theta_pend).*2.0+THE_Psi_pend_D.*THE_Theta_pend_D.*cos(THE_Theta_pend).*sin(THE_Phi_pend).*sin(THE_Psi_pend).*2.0))./2.0-Lz_pend.*(-THE_Phi_D.*cos(THE_Phi).*cos(THE_Psi)+THE_Psi_D.*sin(THE_Phi).*sin(THE_Psi)-THE_Phi_D.*sin(THE_Phi).*sin(THE_Psi).*sin(THE_Theta)+THE_Psi_D.*cos(THE_Phi).*cos(THE_Psi).*sin(THE_Theta)+THE_Theta_D.*cos(THE_Phi).*cos(THE_Theta).*sin(THE_Psi)).*(-THE_Psi_pend_D.*cos(THE_Phi_pend).*cos(THE_Psi_pend)+THE_Phi_pend_D.*sin(THE_Phi_pend).*sin(THE_Psi_pend)-THE_Psi_pend_D.*sin(THE_Phi_pend).*sin(THE_Psi_pend).*sin(THE_Theta_pend)+THE_Phi_pend_D.*cos(THE_Phi_pend).*cos(THE_Psi_pend).*sin(THE_Theta_pend)+THE_Theta_pend_D.*cos(THE_Psi_pend).*cos(THE_Theta_pend).*sin(THE_Phi_pend))+(Lz_pend.*cos(THE_Phi).*cos(THE_Theta).*(THE_Phi_pend_D.^2.*sin(THE_Phi_pend).*sin(THE_Psi_pend)+THE_Psi_pend_D.^2.*sin(THE_Phi_pend).*sin(THE_Psi_pend)+THE_Phi_pend_D.^2.*cos(THE_Phi_pend).*cos(THE_Psi_pend).*sin(THE_Theta_pend)+THE_Psi_pend_D.^2.*cos(THE_Phi_pend).*cos(THE_Psi_pend).*sin(THE_Theta_pend)+THE_Theta_pend_D.^2.*cos(THE_Phi_pend).*cos(THE_Psi_pend).*sin(THE_Theta_pend)-THE_Phi_pend_D.*THE_Psi_pend_D.*cos(THE_Phi_pend).*cos(THE_Psi_pend).*2.0+THE_Phi_pend_D.*THE_Theta_pend_D.*cos(THE_Psi_pend).*cos(THE_Theta_pend).*sin(THE_Phi_pend).*2.0+THE_Psi_pend_D.*THE_Theta_pend_D.*cos(THE_Phi_pend).*cos(THE_Theta_pend).*sin(THE_Psi_pend).*2.0-THE_Phi_pend_D.*THE_Psi_pend_D.*sin(THE_Phi_pend).*sin(THE_Psi_pend).*sin(THE_Theta_pend).*2.0))./2.0+Lz_pend.*THE_Phi_D.*cos(THE_Theta).*sin(THE_Phi).*(THE_Phi_pend_D.*cos(THE_Phi_pend).*sin(THE_Psi_pend)+THE_Psi_pend_D.*cos(THE_Psi_pend).*sin(THE_Phi_pend)+THE_Theta_pend_D.*cos(THE_Phi_pend).*cos(THE_Psi_pend).*cos(THE_Theta_pend)-THE_Phi_pend_D.*cos(THE_Psi_pend).*sin(THE_Phi_pend).*sin(THE_Theta_pend)-THE_Psi_pend_D.*cos(THE_Phi_pend).*sin(THE_Psi_pend).*sin(THE_Theta_pend))+Lz_pend.*THE_Theta_D.*cos(THE_Phi).*sin(THE_Theta).*(THE_Phi_pend_D.*cos(THE_Phi_pend).*sin(THE_Psi_pend)+THE_Psi_pend_D.*cos(THE_Psi_pend).*sin(THE_Phi_pend)+THE_Theta_pend_D.*cos(THE_Phi_pend).*cos(THE_Psi_pend).*cos(THE_Theta_pend)-THE_Phi_pend_D.*cos(THE_Psi_pend).*sin(THE_Phi_pend).*sin(THE_Theta_pend)-THE_Psi_pend_D.*cos(THE_Phi_pend).*sin(THE_Psi_pend).*sin(THE_Theta_pend))+(Lz_pend.*THE_Phi_D.^2.*cos(THE_Phi).*cos(THE_Theta).*(sin(THE_Phi_pend).*sin(THE_Psi_pend)+cos(THE_Phi_pend).*cos(THE_Psi_pend).*sin(THE_Theta_pend)))./2.0+(Lz_pend.*THE_Theta_D.^2.*cos(THE_Phi).*cos(THE_Theta).*(sin(THE_Phi_pend).*sin(THE_Psi_pend)+cos(THE_Phi_pend).*cos(THE_Psi_pend).*sin(THE_Theta_pend)))./2.0-Lz_pend.*THE_Phi_D.*THE_Theta_D.*sin(THE_Phi).*sin(THE_Theta).*(sin(THE_Phi_pend).*sin(THE_Psi_pend)+cos(THE_Phi_pend).*cos(THE_Psi_pend).*sin(THE_Theta_pend)))+m_pend.*((Lz_pend.*(cos(THE_Psi).*sin(THE_Phi)-cos(THE_Phi).*sin(THE_Psi).*sin(THE_Theta)).*(cos(THE_Phi_pend).*cos(THE_Psi_pend)+sin(THE_Phi_pend).*sin(THE_Psi_pend).*sin(THE_Theta_pend)))./2.0+(Lz_pend.*cos(THE_Phi).*cos(THE_Theta).*(cos(THE_Psi_pend).*sin(THE_Phi_pend)-cos(THE_Phi_pend).*sin(THE_Psi_pend).*sin(THE_Theta_pend)))./2.0-(Lz_pend.*cos(THE_Theta_pend).*sin(THE_Psi_pend).*(sin(THE_Phi).*sin(THE_Psi)+cos(THE_Phi).*cos(THE_Psi).*sin(THE_Theta)))./2.0).*(((Tv_Z_pend+(Lz_pend.*cos(THE_Psi_pend).*cos(THE_Theta_pend))./2.0).*(THE_Phi_D.^2.*sin(THE_Phi).*sin(THE_Psi)+THE_Psi_D.^2.*sin(THE_Phi).*sin(THE_Psi)+THE_Phi_D.^2.*cos(THE_Phi).*cos(THE_Psi).*sin(THE_Theta)+THE_Psi_D.^2.*cos(THE_Phi).*cos(THE_Psi).*sin(THE_Theta)+THE_Theta_D.^2.*cos(THE_Phi).*cos(THE_Psi).*sin(THE_Theta)-THE_Phi_D.*THE_Psi_D.*cos(THE_Phi).*cos(THE_Psi).*2.0+THE_Phi_D.*THE_Theta_D.*cos(THE_Psi).*cos(THE_Theta).*sin(THE_Phi).*2.0+THE_Psi_D.*THE_Theta_D.*cos(THE_Phi).*cos(THE_Theta).*sin(THE_Psi).*2.0-THE_Phi_D.*THE_Psi_D.*sin(THE_Phi).*sin(THE_Psi).*sin(THE_Theta).*2.0))./2.0+((sin(THE_Phi).*sin(THE_Psi)+cos(THE_Phi).*cos(THE_Psi).*sin(THE_Theta)).*((Lz_pend.*THE_Psi_pend_D.^2.*cos(THE_Psi_pend).*cos(THE_Theta_pend))./2.0+(Lz_pend.*THE_Theta_pend_D.^2.*cos(THE_Psi_pend).*cos(THE_Theta_pend))./2.0-Lz_pend.*THE_Psi_pend_D.*THE_Theta_pend_D.*sin(THE_Psi_pend).*sin(THE_Theta_pend)))./2.0+((Lz_pend.*THE_Psi_pend_D.*cos(THE_Theta_pend).*sin(THE_Psi_pend))./2.0+(Lz_pend.*THE_Theta_pend_D.*cos(THE_Psi_pend).*sin(THE_Theta_pend))./2.0).*(THE_Phi_D.*cos(THE_Phi).*sin(THE_Psi)+THE_Psi_D.*cos(THE_Psi).*sin(THE_Phi)+THE_Theta_D.*cos(THE_Phi).*cos(THE_Psi).*cos(THE_Theta)-THE_Phi_D.*cos(THE_Psi).*sin(THE_Phi).*sin(THE_Theta)-THE_Psi_D.*cos(THE_Phi).*sin(THE_Psi).*sin(THE_Theta))-(Lz_pend.*(cos(THE_Phi_pend).*sin(THE_Psi_pend)-cos(THE_Psi_pend).*sin(THE_Phi_pend).*sin(THE_Theta_pend)).*(-THE_Phi_D.^2.*cos(THE_Psi).*sin(THE_Phi)-THE_Psi_D.^2.*cos(THE_Psi).*sin(THE_Phi)+THE_Phi_D.^2.*cos(THE_Phi).*sin(THE_Psi).*sin(THE_Theta)+THE_Psi_D.^2.*cos(THE_Phi).*sin(THE_Psi).*sin(THE_Theta)+THE_Theta_D.^2.*cos(THE_Phi).*sin(THE_Psi).*sin(THE_Theta)-THE_Phi_D.*THE_Psi_D.*cos(THE_Phi).*sin(THE_Psi).*2.0-THE_Psi_D.*THE_Theta_D.*cos(THE_Phi).*cos(THE_Psi).*cos(THE_Theta).*2.0+THE_Phi_D.*THE_Psi_D.*cos(THE_Psi).*sin(THE_Phi).*sin(THE_Theta).*2.0+THE_Phi_D.*THE_Theta_D.*cos(THE_Theta).*sin(THE_Phi).*sin(THE_Psi).*2.0))./4.0-(Lz_pend.*(cos(THE_Psi).*sin(THE_Phi)-cos(THE_Phi).*sin(THE_Psi).*sin(THE_Theta)).*(-THE_Phi_pend_D.^2.*cos(THE_Phi_pend).*sin(THE_Psi_pend)-THE_Psi_pend_D.^2.*cos(THE_Phi_pend).*sin(THE_Psi_pend)+THE_Phi_pend_D.^2.*cos(THE_Psi_pend).*sin(THE_Phi_pend).*sin(THE_Theta_pend)+THE_Psi_pend_D.^2.*cos(THE_Psi_pend).*sin(THE_Phi_pend).*sin(THE_Theta_pend)+THE_Theta_pend_D.^2.*cos(THE_Psi_pend).*sin(THE_Phi_pend).*sin(THE_Theta_pend)-THE_Phi_pend_D.*THE_Psi_pend_D.*cos(THE_Psi_pend).*sin(THE_Phi_pend).*2.0-THE_Phi_pend_D.*THE_Theta_pend_D.*cos(THE_Phi_pend).*cos(THE_Psi_pend).*cos(THE_Theta_pend).*2.0+THE_Phi_pend_D.*THE_Psi_pend_D.*cos(THE_Phi_pend).*sin(THE_Psi_pend).*sin(THE_Theta_pend).*2.0+THE_Psi_pend_D.*THE_Theta_pend_D.*cos(THE_Theta_pend).*sin(THE_Phi_pend).*sin(THE_Psi_pend).*2.0))./4.0-(Lz_pend.*(-THE_Phi_D.*cos(THE_Phi).*cos(THE_Psi)+THE_Psi_D.*sin(THE_Phi).*sin(THE_Psi)-THE_Phi_D.*sin(THE_Phi).*sin(THE_Psi).*sin(THE_Theta)+THE_Psi_D.*cos(THE_Phi).*cos(THE_Psi).*sin(THE_Theta)+THE_Theta_D.*cos(THE_Phi).*cos(THE_Theta).*sin(THE_Psi)).*(-THE_Psi_pend_D.*cos(THE_Phi_pend).*cos(THE_Psi_pend)+THE_Phi_pend_D.*sin(THE_Phi_pend).*sin(THE_Psi_pend)-THE_Psi_pend_D.*sin(THE_Phi_pend).*sin(THE_Psi_pend).*sin(THE_Theta_pend)+THE_Phi_pend_D.*cos(THE_Phi_pend).*cos(THE_Psi_pend).*sin(THE_Theta_pend)+THE_Theta_pend_D.*cos(THE_Psi_pend).*cos(THE_Theta_pend).*sin(THE_Phi_pend)))./2.0+(Lz_pend.*cos(THE_Phi).*cos(THE_Theta).*(THE_Phi_pend_D.^2.*sin(THE_Phi_pend).*sin(THE_Psi_pend)+THE_Psi_pend_D.^2.*sin(THE_Phi_pend).*sin(THE_Psi_pend)+THE_Phi_pend_D.^2.*cos(THE_Phi_pend).*cos(THE_Psi_pend).*sin(THE_Theta_pend)+THE_Psi_pend_D.^2.*cos(THE_Phi_pend).*cos(THE_Psi_pend).*sin(THE_Theta_pend)+THE_Theta_pend_D.^2.*cos(THE_Phi_pend).*cos(THE_Psi_pend).*sin(THE_Theta_pend)-THE_Phi_pend_D.*THE_Psi_pend_D.*cos(THE_Phi_pend).*cos(THE_Psi_pend).*2.0+THE_Phi_pend_D.*THE_Theta_pend_D.*cos(THE_Psi_pend).*cos(THE_Theta_pend).*sin(THE_Phi_pend).*2.0+THE_Psi_pend_D.*THE_Theta_pend_D.*cos(THE_Phi_pend).*cos(THE_Theta_pend).*sin(THE_Psi_pend).*2.0-THE_Phi_pend_D.*THE_Psi_pend_D.*sin(THE_Phi_pend).*sin(THE_Psi_pend).*sin(THE_Theta_pend).*2.0))./4.0+(Lz_pend.*THE_Phi_D.*cos(THE_Theta).*sin(THE_Phi).*(THE_Phi_pend_D.*cos(THE_Phi_pend).*sin(THE_Psi_pend)+THE_Psi_pend_D.*cos(THE_Psi_pend).*sin(THE_Phi_pend)+THE_Theta_pend_D.*cos(THE_Phi_pend).*cos(THE_Psi_pend).*cos(THE_Theta_pend)-THE_Phi_pend_D.*cos(THE_Psi_pend).*sin(THE_Phi_pend).*sin(THE_Theta_pend)-THE_Psi_pend_D.*cos(THE_Phi_pend).*sin(THE_Psi_pend).*sin(THE_Theta_pend)))./2.0+(Lz_pend.*THE_Theta_D.*cos(THE_Phi).*sin(THE_Theta).*(THE_Phi_pend_D.*cos(THE_Phi_pend).*sin(THE_Psi_pend)+THE_Psi_pend_D.*cos(THE_Psi_pend).*sin(THE_Phi_pend)+THE_Theta_pend_D.*cos(THE_Phi_pend).*cos(THE_Psi_pend).*cos(THE_Theta_pend)-THE_Phi_pend_D.*cos(THE_Psi_pend).*sin(THE_Phi_pend).*sin(THE_Theta_pend)-THE_Psi_pend_D.*cos(THE_Phi_pend).*sin(THE_Psi_pend).*sin(THE_Theta_pend)))./2.0+(Lz_pend.*THE_Phi_D.^2.*cos(THE_Phi).*cos(THE_Theta).*(sin(THE_Phi_pend).*sin(THE_Psi_pend)+cos(THE_Phi_pend).*cos(THE_Psi_pend).*sin(THE_Theta_pend)))./4.0+(Lz_pend.*THE_Theta_D.^2.*cos(THE_Phi).*cos(THE_Theta).*(sin(THE_Phi_pend).*sin(THE_Psi_pend)+cos(THE_Phi_pend).*cos(THE_Psi_pend).*sin(THE_Theta_pend)))./4.0-(Lz_pend.*THE_Phi_D.*THE_Theta_D.*sin(THE_Phi).*sin(THE_Theta).*(sin(THE_Phi_pend).*sin(THE_Psi_pend)+cos(THE_Phi_pend).*cos(THE_Psi_pend).*sin(THE_Theta_pend)))./2.0)+m_pend.*(-THE_Z_D+(Lz_pend.*sin(THE_Theta).*(THE_Phi_pend_D.*cos(THE_Phi_pend).*sin(THE_Psi_pend)+THE_Psi_pend_D.*cos(THE_Psi_pend).*sin(THE_Phi_pend)+THE_Theta_pend_D.*cos(THE_Phi_pend).*cos(THE_Psi_pend).*cos(THE_Theta_pend)-THE_Phi_pend_D.*cos(THE_Psi_pend).*sin(THE_Phi_pend).*sin(THE_Theta_pend)-THE_Psi_pend_D.*cos(THE_Phi_pend).*sin(THE_Psi_pend).*sin(THE_Theta_pend)))./2.0+cos(THE_Psi).*cos(THE_Theta).*((Lz_pend.*THE_Psi_pend_D.*cos(THE_Theta_pend).*sin(THE_Psi_pend))./2.0+(Lz_pend.*THE_Theta_pend_D.*cos(THE_Psi_pend).*sin(THE_Theta_pend))./2.0)+THE_Psi_D.*cos(THE_Theta).*sin(THE_Psi).*(Tv_Z_pend+(Lz_pend.*cos(THE_Psi_pend).*cos(THE_Theta_pend))./2.0)+THE_Theta_D.*cos(THE_Psi).*sin(THE_Theta).*(Tv_Z_pend+(Lz_pend.*cos(THE_Psi_pend).*cos(THE_Theta_pend))./2.0)+(Lz_pend.*THE_Theta_D.*cos(THE_Theta).*(sin(THE_Phi_pend).*sin(THE_Psi_pend)+cos(THE_Phi_pend).*cos(THE_Psi_pend).*sin(THE_Theta_pend)))./2.0-(Lz_pend.*cos(THE_Theta).*sin(THE_Psi).*(-THE_Psi_pend_D.*cos(THE_Phi_pend).*cos(THE_Psi_pend)+THE_Phi_pend_D.*sin(THE_Phi_pend).*sin(THE_Psi_pend)-THE_Psi_pend_D.*sin(THE_Phi_pend).*sin(THE_Psi_pend).*sin(THE_Theta_pend)+THE_Phi_pend_D.*cos(THE_Phi_pend).*cos(THE_Psi_pend).*sin(THE_Theta_pend)+THE_Theta_pend_D.*cos(THE_Psi_pend).*cos(THE_Theta_pend).*sin(THE_Phi_pend)))./2.0+(Lz_pend.*THE_Psi_D.*cos(THE_Psi).*cos(THE_Theta).*(cos(THE_Phi_pend).*sin(THE_Psi_pend)-cos(THE_Psi_pend).*sin(THE_Phi_pend).*sin(THE_Theta_pend)))./2.0-(Lz_pend.*THE_Theta_D.*sin(THE_Psi).*sin(THE_Theta).*(cos(THE_Phi_pend).*sin(THE_Psi_pend)-cos(THE_Psi_pend).*sin(THE_Phi_pend).*sin(THE_Theta_pend)))./2.0).*((Lz_pend.*sin(THE_Theta).*(-THE_Phi_pend_D.*cos(THE_Phi_pend).*cos(THE_Psi_pend)+THE_Psi_pend_D.*sin(THE_Phi_pend).*sin(THE_Psi_pend)-THE_Phi_pend_D.*sin(THE_Phi_pend).*sin(THE_Psi_pend).*sin(THE_Theta_pend)+THE_Psi_pend_D.*cos(THE_Phi_pend).*cos(THE_Psi_pend).*sin(THE_Theta_pend)+THE_Theta_pend_D.*cos(THE_Phi_pend).*cos(THE_Theta_pend).*sin(THE_Psi_pend)))./4.0-(Lz_pend.*THE_Theta_D.*cos(THE_Theta).*(cos(THE_Psi_pend).*sin(THE_Phi_pend)-cos(THE_Phi_pend).*sin(THE_Psi_pend).*sin(THE_Theta_pend)))./4.0-(Lz_pend.*cos(THE_Theta).*sin(THE_Psi).*(-THE_Phi_pend_D.*cos(THE_Psi_pend).*sin(THE_Phi_pend)-THE_Psi_pend_D.*cos(THE_Phi_pend).*sin(THE_Psi_pend)+THE_Phi_pend_D.*cos(THE_Phi_pend).*sin(THE_Psi_pend).*sin(THE_Theta_pend)+THE_Psi_pend_D.*cos(THE_Psi_pend).*sin(THE_Phi_pend).*sin(THE_Theta_pend)+THE_Theta_pend_D.*cos(THE_Theta_pend).*sin(THE_Phi_pend).*sin(THE_Psi_pend)))./4.0-(Lz_pend.*THE_Psi_D.*cos(THE_Psi).*cos(THE_Theta).*(cos(THE_Phi_pend).*cos(THE_Psi_pend)+sin(THE_Phi_pend).*sin(THE_Psi_pend).*sin(THE_Theta_pend)))./4.0+(Lz_pend.*THE_Theta_D.*sin(THE_Psi).*sin(THE_Theta).*(cos(THE_Phi_pend).*cos(THE_Psi_pend)+sin(THE_Phi_pend).*sin(THE_Psi_pend).*sin(THE_Theta_pend)))./4.0-(Lz_pend.*THE_Psi_pend_D.*cos(THE_Psi).*cos(THE_Theta).*cos(THE_Psi_pend).*cos(THE_Theta_pend))./4.0+(Lz_pend.*THE_Psi_D.*cos(THE_Theta).*cos(THE_Theta_pend).*sin(THE_Psi).*sin(THE_Psi_pend))./4.0+(Lz_pend.*THE_Theta_D.*cos(THE_Psi).*cos(THE_Theta_pend).*sin(THE_Theta).*sin(THE_Psi_pend))./4.0+(Lz_pend.*THE_Theta_pend_D.*cos(THE_Psi).*cos(THE_Theta).*sin(THE_Psi_pend).*sin(THE_Theta_pend))./4.0)+m_pend.*(THE_Z_D.*(-1.0./2.0)+(Lz_pend.*sin(THE_Theta).*(THE_Phi_pend_D.*cos(THE_Phi_pend).*sin(THE_Psi_pend)+THE_Psi_pend_D.*cos(THE_Psi_pend).*sin(THE_Phi_pend)+THE_Theta_pend_D.*cos(THE_Phi_pend).*cos(THE_Psi_pend).*cos(THE_Theta_pend)-THE_Phi_pend_D.*cos(THE_Psi_pend).*sin(THE_Phi_pend).*sin(THE_Theta_pend)-THE_Psi_pend_D.*cos(THE_Phi_pend).*sin(THE_Psi_pend).*sin(THE_Theta_pend)))./4.0+(cos(THE_Psi).*cos(THE_Theta).*((Lz_pend.*THE_Psi_pend_D.*cos(THE_Theta_pend).*sin(THE_Psi_pend))./2.0+(Lz_pend.*THE_Theta_pend_D.*cos(THE_Psi_pend).*sin(THE_Theta_pend))./2.0))./2.0+(THE_Psi_D.*cos(THE_Theta).*sin(THE_Psi).*(Tv_Z_pend+(Lz_pend.*cos(THE_Psi_pend).*cos(THE_Theta_pend))./2.0))./2.0+(THE_Theta_D.*cos(THE_Psi).*sin(THE_Theta).*(Tv_Z_pend+(Lz_pend.*cos(THE_Psi_pend).*cos(THE_Theta_pend))./2.0))./2.0+(Lz_pend.*THE_Theta_D.*cos(THE_Theta).*(sin(THE_Phi_pend).*sin(THE_Psi_pend)+cos(THE_Phi_pend).*cos(THE_Psi_pend).*sin(THE_Theta_pend)))./4.0-(Lz_pend.*cos(THE_Theta).*sin(THE_Psi).*(-THE_Psi_pend_D.*cos(THE_Phi_pend).*cos(THE_Psi_pend)+THE_Phi_pend_D.*sin(THE_Phi_pend).*sin(THE_Psi_pend)-THE_Psi_pend_D.*sin(THE_Phi_pend).*sin(THE_Psi_pend).*sin(THE_Theta_pend)+THE_Phi_pend_D.*cos(THE_Phi_pend).*cos(THE_Psi_pend).*sin(THE_Theta_pend)+THE_Theta_pend_D.*cos(THE_Psi_pend).*cos(THE_Theta_pend).*sin(THE_Phi_pend)))./4.0+(Lz_pend.*THE_Psi_D.*cos(THE_Psi).*cos(THE_Theta).*(cos(THE_Phi_pend).*sin(THE_Psi_pend)-cos(THE_Psi_pend).*sin(THE_Phi_pend).*sin(THE_Theta_pend)))./4.0-(Lz_pend.*THE_Theta_D.*sin(THE_Psi).*sin(THE_Theta).*(cos(THE_Phi_pend).*sin(THE_Psi_pend)-cos(THE_Psi_pend).*sin(THE_Phi_pend).*sin(THE_Theta_pend)))./4.0).*((Lz_pend.*sin(THE_Theta).*(-THE_Phi_pend_D.*cos(THE_Phi_pend).*cos(THE_Psi_pend)+THE_Psi_pend_D.*sin(THE_Phi_pend).*sin(THE_Psi_pend)-THE_Phi_pend_D.*sin(THE_Phi_pend).*sin(THE_Psi_pend).*sin(THE_Theta_pend)+THE_Psi_pend_D.*cos(THE_Phi_pend).*cos(THE_Psi_pend).*sin(THE_Theta_pend)+THE_Theta_pend_D.*cos(THE_Phi_pend).*cos(THE_Theta_pend).*sin(THE_Psi_pend)))./2.0-(Lz_pend.*THE_Theta_D.*cos(THE_Theta).*(cos(THE_Psi_pend).*sin(THE_Phi_pend)-cos(THE_Phi_pend).*sin(THE_Psi_pend).*sin(THE_Theta_pend)))./2.0-(Lz_pend.*cos(THE_Theta).*sin(THE_Psi).*(-THE_Phi_pend_D.*cos(THE_Psi_pend).*sin(THE_Phi_pend)-THE_Psi_pend_D.*cos(THE_Phi_pend).*sin(THE_Psi_pend)+THE_Phi_pend_D.*cos(THE_Phi_pend).*sin(THE_Psi_pend).*sin(THE_Theta_pend)+THE_Psi_pend_D.*cos(THE_Psi_pend).*sin(THE_Phi_pend).*sin(THE_Theta_pend)+THE_Theta_pend_D.*cos(THE_Theta_pend).*sin(THE_Phi_pend).*sin(THE_Psi_pend)))./2.0-(Lz_pend.*THE_Psi_D.*cos(THE_Psi).*cos(THE_Theta).*(cos(THE_Phi_pend).*cos(THE_Psi_pend)+sin(THE_Phi_pend).*sin(THE_Psi_pend).*sin(THE_Theta_pend)))./2.0+(Lz_pend.*THE_Theta_D.*sin(THE_Psi).*sin(THE_Theta).*(cos(THE_Phi_pend).*cos(THE_Psi_pend)+sin(THE_Phi_pend).*sin(THE_Psi_pend).*sin(THE_Theta_pend)))./2.0-(Lz_pend.*THE_Psi_pend_D.*cos(THE_Psi).*cos(THE_Theta).*cos(THE_Psi_pend).*cos(THE_Theta_pend))./2.0+(Lz_pend.*THE_Psi_D.*cos(THE_Theta).*cos(THE_Theta_pend).*sin(THE_Psi).*sin(THE_Psi_pend))./2.0+(Lz_pend.*THE_Theta_D.*cos(THE_Psi).*cos(THE_Theta_pend).*sin(THE_Theta).*sin(THE_Psi_pend))./2.0+(Lz_pend.*THE_Theta_pend_D.*cos(THE_Psi).*cos(THE_Theta).*sin(THE_Psi_pend).*sin(THE_Theta_pend))./2.0)+m_pend.*((((Lz_pend.*THE_Psi_pend_D.*cos(THE_Psi_pend).*cos(THE_Theta_pend))./2.0-(Lz_pend.*THE_Theta_pend_D.*sin(THE_Psi_pend).*sin(THE_Theta_pend))./2.0).*(sin(THE_Phi).*sin(THE_Psi)+cos(THE_Phi).*cos(THE_Psi).*sin(THE_Theta)))./2.0+(Lz_pend.*(cos(THE_Phi_pend).*cos(THE_Psi_pend)+sin(THE_Phi_pend).*sin(THE_Psi_pend).*sin(THE_Theta_pend)).*(-THE_Phi_D.*cos(THE_Phi).*cos(THE_Psi)+THE_Psi_D.*sin(THE_Phi).*sin(THE_Psi)-THE_Phi_D.*sin(THE_Phi).*sin(THE_Psi).*sin(THE_Theta)+THE_Psi_D.*cos(THE_Phi).*cos(THE_Psi).*sin(THE_Theta)+THE_Theta_D.*cos(THE_Phi).*cos(THE_Theta).*sin(THE_Psi)))./4.0-(Lz_pend.*(cos(THE_Psi).*sin(THE_Phi)-cos(THE_Phi).*sin(THE_Psi).*sin(THE_Theta)).*(-THE_Phi_pend_D.*cos(THE_Psi_pend).*sin(THE_Phi_pend)-THE_Psi_pend_D.*cos(THE_Phi_pend).*sin(THE_Psi_pend)+THE_Phi_pend_D.*cos(THE_Phi_pend).*sin(THE_Psi_pend).*sin(THE_Theta_pend)+THE_Psi_pend_D.*cos(THE_Psi_pend).*sin(THE_Phi_pend).*sin(THE_Theta_pend)+THE_Theta_pend_D.*cos(THE_Theta_pend).*sin(THE_Phi_pend).*sin(THE_Psi_pend)))./4.0+(Lz_pend.*cos(THE_Theta_pend).*sin(THE_Psi_pend).*(THE_Phi_D.*cos(THE_Phi).*sin(THE_Psi)+THE_Psi_D.*cos(THE_Psi).*sin(THE_Phi)+THE_Theta_D.*cos(THE_Phi).*cos(THE_Psi).*cos(THE_Theta)-THE_Phi_D.*cos(THE_Psi).*sin(THE_Phi).*sin(THE_Theta)-THE_Psi_D.*cos(THE_Phi).*sin(THE_Psi).*sin(THE_Theta)))./4.0+(Lz_pend.*cos(THE_Phi).*cos(THE_Theta).*(-THE_Phi_pend_D.*cos(THE_Phi_pend).*cos(THE_Psi_pend)+THE_Psi_pend_D.*sin(THE_Phi_pend).*sin(THE_Psi_pend)-THE_Phi_pend_D.*sin(THE_Phi_pend).*sin(THE_Psi_pend).*sin(THE_Theta_pend)+THE_Psi_pend_D.*cos(THE_Phi_pend).*cos(THE_Psi_pend).*sin(THE_Theta_pend)+THE_Theta_pend_D.*cos(THE_Phi_pend).*cos(THE_Theta_pend).*sin(THE_Psi_pend)))./4.0+(Lz_pend.*THE_Phi_D.*cos(THE_Theta).*sin(THE_Phi).*(cos(THE_Psi_pend).*sin(THE_Phi_pend)-cos(THE_Phi_pend).*sin(THE_Psi_pend).*sin(THE_Theta_pend)))./4.0+(Lz_pend.*THE_Theta_D.*cos(THE_Phi).*sin(THE_Theta).*(cos(THE_Psi_pend).*sin(THE_Phi_pend)-cos(THE_Phi_pend).*sin(THE_Psi_pend).*sin(THE_Theta_pend)))./4.0).*(-THE_X_D+((Lz_pend.*THE_Psi_pend_D.*cos(THE_Theta_pend).*sin(THE_Psi_pend))./2.0+(Lz_pend.*THE_Theta_pend_D.*cos(THE_Psi_pend).*sin(THE_Theta_pend))./2.0).*(sin(THE_Phi).*sin(THE_Psi)+cos(THE_Phi).*cos(THE_Psi).*sin(THE_Theta))-(Tv_Z_pend+(Lz_pend.*cos(THE_Psi_pend).*cos(THE_Theta_pend))./2.0).*(THE_Phi_D.*cos(THE_Phi).*sin(THE_Psi)+THE_Psi_D.*cos(THE_Psi).*sin(THE_Phi)+THE_Theta_D.*cos(THE_Phi).*cos(THE_Psi).*cos(THE_Theta)-THE_Phi_D.*cos(THE_Psi).*sin(THE_Phi).*sin(THE_Theta)-THE_Psi_D.*cos(THE_Phi).*sin(THE_Psi).*sin(THE_Theta))+(Lz_pend.*(cos(THE_Phi_pend).*sin(THE_Psi_pend)-cos(THE_Psi_pend).*sin(THE_Phi_pend).*sin(THE_Theta_pend)).*(-THE_Phi_D.*cos(THE_Phi).*cos(THE_Psi)+THE_Psi_D.*sin(THE_Phi).*sin(THE_Psi)-THE_Phi_D.*sin(THE_Phi).*sin(THE_Psi).*sin(THE_Theta)+THE_Psi_D.*cos(THE_Phi).*cos(THE_Psi).*sin(THE_Theta)+THE_Theta_D.*cos(THE_Phi).*cos(THE_Theta).*sin(THE_Psi)))./2.0+(Lz_pend.*(cos(THE_Psi).*sin(THE_Phi)-cos(THE_Phi).*sin(THE_Psi).*sin(THE_Theta)).*(-THE_Psi_pend_D.*cos(THE_Phi_pend).*cos(THE_Psi_pend)+THE_Phi_pend_D.*sin(THE_Phi_pend).*sin(THE_Psi_pend)-THE_Psi_pend_D.*sin(THE_Phi_pend).*sin(THE_Psi_pend).*sin(THE_Theta_pend)+THE_Phi_pend_D.*cos(THE_Phi_pend).*cos(THE_Psi_pend).*sin(THE_Theta_pend)+THE_Theta_pend_D.*cos(THE_Psi_pend).*cos(THE_Theta_pend).*sin(THE_Phi_pend)))./2.0-(Lz_pend.*cos(THE_Phi).*cos(THE_Theta).*(THE_Phi_pend_D.*cos(THE_Phi_pend).*sin(THE_Psi_pend)+THE_Psi_pend_D.*cos(THE_Psi_pend).*sin(THE_Phi_pend)+THE_Theta_pend_D.*cos(THE_Phi_pend).*cos(THE_Psi_pend).*cos(THE_Theta_pend)-THE_Phi_pend_D.*cos(THE_Psi_pend).*sin(THE_Phi_pend).*sin(THE_Theta_pend)-THE_Psi_pend_D.*cos(THE_Phi_pend).*sin(THE_Psi_pend).*sin(THE_Theta_pend)))./2.0+(Lz_pend.*THE_Phi_D.*cos(THE_Theta).*sin(THE_Phi).*(sin(THE_Phi_pend).*sin(THE_Psi_pend)+cos(THE_Phi_pend).*cos(THE_Psi_pend).*sin(THE_Theta_pend)))./2.0+(Lz_pend.*THE_Theta_D.*cos(THE_Phi).*sin(THE_Theta).*(sin(THE_Phi_pend).*sin(THE_Psi_pend)+cos(THE_Phi_pend).*cos(THE_Psi_pend).*sin(THE_Theta_pend)))./2.0)+m_pend.*(((Lz_pend.*THE_Psi_pend_D.*cos(THE_Psi_pend).*cos(THE_Theta_pend))./2.0-(Lz_pend.*THE_Theta_pend_D.*sin(THE_Psi_pend).*sin(THE_Theta_pend))./2.0).*(sin(THE_Phi).*sin(THE_Psi)+cos(THE_Phi).*cos(THE_Psi).*sin(THE_Theta))+(Lz_pend.*(cos(THE_Phi_pend).*cos(THE_Psi_pend)+sin(THE_Phi_pend).*sin(THE_Psi_pend).*sin(THE_Theta_pend)).*(-THE_Phi_D.*cos(THE_Phi).*cos(THE_Psi)+THE_Psi_D.*sin(THE_Phi).*sin(THE_Psi)-THE_Phi_D.*sin(THE_Phi).*sin(THE_Psi).*sin(THE_Theta)+THE_Psi_D.*cos(THE_Phi).*cos(THE_Psi).*sin(THE_Theta)+THE_Theta_D.*cos(THE_Phi).*cos(THE_Theta).*sin(THE_Psi)))./2.0-(Lz_pend.*(cos(THE_Psi).*sin(THE_Phi)-cos(THE_Phi).*sin(THE_Psi).*sin(THE_Theta)).*(-THE_Phi_pend_D.*cos(THE_Psi_pend).*sin(THE_Phi_pend)-THE_Psi_pend_D.*cos(THE_Phi_pend).*sin(THE_Psi_pend)+THE_Phi_pend_D.*cos(THE_Phi_pend).*sin(THE_Psi_pend).*sin(THE_Theta_pend)+THE_Psi_pend_D.*cos(THE_Psi_pend).*sin(THE_Phi_pend).*sin(THE_Theta_pend)+THE_Theta_pend_D.*cos(THE_Theta_pend).*sin(THE_Phi_pend).*sin(THE_Psi_pend)))./2.0+(Lz_pend.*cos(THE_Theta_pend).*sin(THE_Psi_pend).*(THE_Phi_D.*cos(THE_Phi).*sin(THE_Psi)+THE_Psi_D.*cos(THE_Psi).*sin(THE_Phi)+THE_Theta_D.*cos(THE_Phi).*cos(THE_Psi).*cos(THE_Theta)-THE_Phi_D.*cos(THE_Psi).*sin(THE_Phi).*sin(THE_Theta)-THE_Psi_D.*cos(THE_Phi).*sin(THE_Psi).*sin(THE_Theta)))./2.0+(Lz_pend.*cos(THE_Phi).*cos(THE_Theta).*(-THE_Phi_pend_D.*cos(THE_Phi_pend).*cos(THE_Psi_pend)+THE_Psi_pend_D.*sin(THE_Phi_pend).*sin(THE_Psi_pend)-THE_Phi_pend_D.*sin(THE_Phi_pend).*sin(THE_Psi_pend).*sin(THE_Theta_pend)+THE_Psi_pend_D.*cos(THE_Phi_pend).*cos(THE_Psi_pend).*sin(THE_Theta_pend)+THE_Theta_pend_D.*cos(THE_Phi_pend).*cos(THE_Theta_pend).*sin(THE_Psi_pend)))./2.0+(Lz_pend.*THE_Phi_D.*cos(THE_Theta).*sin(THE_Phi).*(cos(THE_Psi_pend).*sin(THE_Phi_pend)-cos(THE_Phi_pend).*sin(THE_Psi_pend).*sin(THE_Theta_pend)))./2.0+(Lz_pend.*THE_Theta_D.*cos(THE_Phi).*sin(THE_Theta).*(cos(THE_Psi_pend).*sin(THE_Phi_pend)-cos(THE_Phi_pend).*sin(THE_Psi_pend).*sin(THE_Theta_pend)))./2.0).*(THE_X_D.*(-1.0./2.0)+(((Lz_pend.*THE_Psi_pend_D.*cos(THE_Theta_pend).*sin(THE_Psi_pend))./2.0+(Lz_pend.*THE_Theta_pend_D.*cos(THE_Psi_pend).*sin(THE_Theta_pend))./2.0).*(sin(THE_Phi).*sin(THE_Psi)+cos(THE_Phi).*cos(THE_Psi).*sin(THE_Theta)))./2.0-((Tv_Z_pend+(Lz_pend.*cos(THE_Psi_pend).*cos(THE_Theta_pend))./2.0).*(THE_Phi_D.*cos(THE_Phi).*sin(THE_Psi)+THE_Psi_D.*cos(THE_Psi).*sin(THE_Phi)+THE_Theta_D.*cos(THE_Phi).*cos(THE_Psi).*cos(THE_Theta)-THE_Phi_D.*cos(THE_Psi).*sin(THE_Phi).*sin(THE_Theta)-THE_Psi_D.*cos(THE_Phi).*sin(THE_Psi).*sin(THE_Theta)))./2.0+(Lz_pend.*(cos(THE_Phi_pend).*sin(THE_Psi_pend)-cos(THE_Psi_pend).*sin(THE_Phi_pend).*sin(THE_Theta_pend)).*(-THE_Phi_D.*cos(THE_Phi).*cos(THE_Psi)+THE_Psi_D.*sin(THE_Phi).*sin(THE_Psi)-THE_Phi_D.*sin(THE_Phi).*sin(THE_Psi).*sin(THE_Theta)+THE_Psi_D.*cos(THE_Phi).*cos(THE_Psi).*sin(THE_Theta)+THE_Theta_D.*cos(THE_Phi).*cos(THE_Theta).*sin(THE_Psi)))./4.0+(Lz_pend.*(cos(THE_Psi).*sin(THE_Phi)-cos(THE_Phi).*sin(THE_Psi).*sin(THE_Theta)).*(-THE_Psi_pend_D.*cos(THE_Phi_pend).*cos(THE_Psi_pend)+THE_Phi_pend_D.*sin(THE_Phi_pend).*sin(THE_Psi_pend)-THE_Psi_pend_D.*sin(THE_Phi_pend).*sin(THE_Psi_pend).*sin(THE_Theta_pend)+THE_Phi_pend_D.*cos(THE_Phi_pend).*cos(THE_Psi_pend).*sin(THE_Theta_pend)+THE_Theta_pend_D.*cos(THE_Psi_pend).*cos(THE_Theta_pend).*sin(THE_Phi_pend)))./4.0-(Lz_pend.*cos(THE_Phi).*cos(THE_Theta).*(THE_Phi_pend_D.*cos(THE_Phi_pend).*sin(THE_Psi_pend)+THE_Psi_pend_D.*cos(THE_Psi_pend).*sin(THE_Phi_pend)+THE_Theta_pend_D.*cos(THE_Phi_pend).*cos(THE_Psi_pend).*cos(THE_Theta_pend)-THE_Phi_pend_D.*cos(THE_Psi_pend).*sin(THE_Phi_pend).*sin(THE_Theta_pend)-THE_Psi_pend_D.*cos(THE_Phi_pend).*sin(THE_Psi_pend).*sin(THE_Theta_pend)))./4.0+(Lz_pend.*THE_Phi_D.*cos(THE_Theta).*sin(THE_Phi).*(sin(THE_Phi_pend).*sin(THE_Psi_pend)+cos(THE_Phi_pend).*cos(THE_Psi_pend).*sin(THE_Theta_pend)))./4.0+(Lz_pend.*THE_Theta_D.*cos(THE_Phi).*sin(THE_Theta).*(sin(THE_Phi_pend).*sin(THE_Psi_pend)+cos(THE_Phi_pend).*cos(THE_Psi_pend).*sin(THE_Theta_pend)))./4.0)-m_pend.*(((Lz_pend.*THE_Psi_pend_D.*cos(THE_Psi_pend).*cos(THE_Theta_pend))./2.0-(Lz_pend.*THE_Theta_pend_D.*sin(THE_Psi_pend).*sin(THE_Theta_pend))./2.0).*(cos(THE_Phi).*sin(THE_Psi)-cos(THE_Psi).*sin(THE_Phi).*sin(THE_Theta)).*(-1.0./2.0)+(Lz_pend.*(cos(THE_Phi_pend).*cos(THE_Psi_pend)+sin(THE_Phi_pend).*sin(THE_Psi_pend).*sin(THE_Theta_pend)).*(-THE_Phi_D.*cos(THE_Psi).*sin(THE_Phi)-THE_Psi_D.*cos(THE_Phi).*sin(THE_Psi)+THE_Phi_D.*cos(THE_Phi).*sin(THE_Psi).*sin(THE_Theta)+THE_Psi_D.*cos(THE_Psi).*sin(THE_Phi).*sin(THE_Theta)+THE_Theta_D.*cos(THE_Theta).*sin(THE_Phi).*sin(THE_Psi)))./4.0+(Lz_pend.*(cos(THE_Phi).*cos(THE_Psi)+sin(THE_Phi).*sin(THE_Psi).*sin(THE_Theta)).*(-THE_Phi_pend_D.*cos(THE_Psi_pend).*sin(THE_Phi_pend)-THE_Psi_pend_D.*cos(THE_Phi_pend).*sin(THE_Psi_pend)+THE_Phi_pend_D.*cos(THE_Phi_pend).*sin(THE_Psi_pend).*sin(THE_Theta_pend)+THE_Psi_pend_D.*cos(THE_Psi_pend).*sin(THE_Phi_pend).*sin(THE_Theta_pend)+THE_Theta_pend_D.*cos(THE_Theta_pend).*sin(THE_Phi_pend).*sin(THE_Psi_pend)))./4.0+(Lz_pend.*cos(THE_Theta_pend).*sin(THE_Psi_pend).*(-THE_Psi_D.*cos(THE_Phi).*cos(THE_Psi)+THE_Phi_D.*sin(THE_Phi).*sin(THE_Psi)-THE_Psi_D.*sin(THE_Phi).*sin(THE_Psi).*sin(THE_Theta)+THE_Phi_D.*cos(THE_Phi).*cos(THE_Psi).*sin(THE_Theta)+THE_Theta_D.*cos(THE_Psi).*cos(THE_Theta).*sin(THE_Phi)))./4.0+(Lz_pend.*cos(THE_Theta).*sin(THE_Phi).*(-THE_Phi_pend_D.*cos(THE_Phi_pend).*cos(THE_Psi_pend)+THE_Psi_pend_D.*sin(THE_Phi_pend).*sin(THE_Psi_pend)-THE_Phi_pend_D.*sin(THE_Phi_pend).*sin(THE_Psi_pend).*sin(THE_Theta_pend)+THE_Psi_pend_D.*cos(THE_Phi_pend).*cos(THE_Psi_pend).*sin(THE_Theta_pend)+THE_Theta_pend_D.*cos(THE_Phi_pend).*cos(THE_Theta_pend).*sin(THE_Psi_pend)))./4.0-(Lz_pend.*THE_Phi_D.*cos(THE_Phi).*cos(THE_Theta).*(cos(THE_Psi_pend).*sin(THE_Phi_pend)-cos(THE_Phi_pend).*sin(THE_Psi_pend).*sin(THE_Theta_pend)))./4.0+(Lz_pend.*THE_Theta_D.*sin(THE_Phi).*sin(THE_Theta).*(cos(THE_Psi_pend).*sin(THE_Phi_pend)-cos(THE_Phi_pend).*sin(THE_Psi_pend).*sin(THE_Theta_pend)))./4.0).*(THE_Y_D+((Lz_pend.*THE_Psi_pend_D.*cos(THE_Theta_pend).*sin(THE_Psi_pend))./2.0+(Lz_pend.*THE_Theta_pend_D.*cos(THE_Psi_pend).*sin(THE_Theta_pend))./2.0).*(cos(THE_Phi).*sin(THE_Psi)-cos(THE_Psi).*sin(THE_Phi).*sin(THE_Theta))+(Tv_Z_pend+(Lz_pend.*cos(THE_Psi_pend).*cos(THE_Theta_pend))./2.0).*(-THE_Psi_D.*cos(THE_Phi).*cos(THE_Psi)+THE_Phi_D.*sin(THE_Phi).*sin(THE_Psi)-THE_Psi_D.*sin(THE_Phi).*sin(THE_Psi).*sin(THE_Theta)+THE_Phi_D.*cos(THE_Phi).*cos(THE_Psi).*sin(THE_Theta)+THE_Theta_D.*cos(THE_Psi).*cos(THE_Theta).*sin(THE_Phi))+(Lz_pend.*(cos(THE_Phi).*cos(THE_Psi)+sin(THE_Phi).*sin(THE_Psi).*sin(THE_Theta)).*(-THE_Psi_pend_D.*cos(THE_Phi_pend).*cos(THE_Psi_pend)+THE_Phi_pend_D.*sin(THE_Phi_pend).*sin(THE_Psi_pend)-THE_Psi_pend_D.*sin(THE_Phi_pend).*sin(THE_Psi_pend).*sin(THE_Theta_pend)+THE_Phi_pend_D.*cos(THE_Phi_pend).*cos(THE_Psi_pend).*sin(THE_Theta_pend)+THE_Theta_pend_D.*cos(THE_Psi_pend).*cos(THE_Theta_pend).*sin(THE_Phi_pend)))./2.0-(Lz_pend.*(cos(THE_Phi_pend).*sin(THE_Psi_pend)-cos(THE_Psi_pend).*sin(THE_Phi_pend).*sin(THE_Theta_pend)).*(-THE_Phi_D.*cos(THE_Psi).*sin(THE_Phi)-THE_Psi_D.*cos(THE_Phi).*sin(THE_Psi)+THE_Phi_D.*cos(THE_Phi).*sin(THE_Psi).*sin(THE_Theta)+THE_Psi_D.*cos(THE_Psi).*sin(THE_Phi).*sin(THE_Theta)+THE_Theta_D.*cos(THE_Theta).*sin(THE_Phi).*sin(THE_Psi)))./2.0+(Lz_pend.*cos(THE_Theta).*sin(THE_Phi).*(THE_Phi_pend_D.*cos(THE_Phi_pend).*sin(THE_Psi_pend)+THE_Psi_pend_D.*cos(THE_Psi_pend).*sin(THE_Phi_pend)+THE_Theta_pend_D.*cos(THE_Phi_pend).*cos(THE_Psi_pend).*cos(THE_Theta_pend)-THE_Phi_pend_D.*cos(THE_Psi_pend).*sin(THE_Phi_pend).*sin(THE_Theta_pend)-THE_Psi_pend_D.*cos(THE_Phi_pend).*sin(THE_Psi_pend).*sin(THE_Theta_pend)))./2.0+(Lz_pend.*THE_Phi_D.*cos(THE_Phi).*cos(THE_Theta).*(sin(THE_Phi_pend).*sin(THE_Psi_pend)+cos(THE_Phi_pend).*cos(THE_Psi_pend).*sin(THE_Theta_pend)))./2.0-(Lz_pend.*THE_Theta_D.*sin(THE_Phi).*sin(THE_Theta).*(sin(THE_Phi_pend).*sin(THE_Psi_pend)+cos(THE_Phi_pend).*cos(THE_Psi_pend).*sin(THE_Theta_pend)))./2.0)+m_pend.*(Lx_pend.^2./1.2e+1+Ly_pend.^2./1.2e+1).*((cos(THE_Phi_pend).*sin(THE_Psi_pend)-cos(THE_Psi_pend).*sin(THE_Phi_pend).*sin(THE_Theta_pend)).*(THE_Theta_D.*cos(THE_Psi)+THE_Phi_D.*cos(THE_Theta).*sin(THE_Psi))-(THE_Psi_D-THE_Phi_D.*sin(THE_Theta)).*(sin(THE_Phi_pend).*sin(THE_Psi_pend)+cos(THE_Phi_pend).*cos(THE_Psi_pend).*sin(THE_Theta_pend))+THE_Theta_pend_D.*sin(THE_Psi_pend)-THE_Phi_pend_D.*cos(THE_Psi_pend).*cos(THE_Theta_pend)+cos(THE_Psi_pend).*cos(THE_Theta_pend).*(THE_Theta_D.*sin(THE_Psi)-THE_Phi_D.*cos(THE_Psi).*cos(THE_Theta))).*(((cos(THE_Phi_pend).*cos(THE_Psi_pend)+sin(THE_Phi_pend).*sin(THE_Psi_pend).*sin(THE_Theta_pend)).*(THE_Theta_D.*cos(THE_Psi)+THE_Phi_D.*cos(THE_Theta).*sin(THE_Psi)))./2.0+(THE_Theta_pend_D.*cos(THE_Psi_pend))./2.0-((THE_Psi_D-THE_Phi_D.*sin(THE_Theta)).*(cos(THE_Psi_pend).*sin(THE_Phi_pend)-cos(THE_Phi_pend).*sin(THE_Psi_pend).*sin(THE_Theta_pend)))./2.0+(THE_Phi_pend_D.*cos(THE_Theta_pend).*sin(THE_Psi_pend))./2.0-(cos(THE_Theta_pend).*sin(THE_Psi_pend).*(THE_Theta_D.*sin(THE_Psi)-THE_Phi_D.*cos(THE_Psi).*cos(THE_Theta)))./2.0)+m_pend.*(Lx_pend.^2./1.2e+1+Ly_pend.^2./1.2e+1).*(((cos(THE_Phi_pend).*sin(THE_Psi_pend)-cos(THE_Psi_pend).*sin(THE_Phi_pend).*sin(THE_Theta_pend)).*(THE_Theta_D.*cos(THE_Psi)+THE_Phi_D.*cos(THE_Theta).*sin(THE_Psi)))./2.0-((THE_Psi_D-THE_Phi_D.*sin(THE_Theta)).*(sin(THE_Phi_pend).*sin(THE_Psi_pend)+cos(THE_Phi_pend).*cos(THE_Psi_pend).*sin(THE_Theta_pend)))./2.0+(THE_Theta_pend_D.*sin(THE_Psi_pend))./2.0-(THE_Phi_pend_D.*cos(THE_Psi_pend).*cos(THE_Theta_pend))./2.0+(cos(THE_Psi_pend).*cos(THE_Theta_pend).*(THE_Theta_D.*sin(THE_Psi)-THE_Phi_D.*cos(THE_Psi).*cos(THE_Theta)))./2.0).*((cos(THE_Phi_pend).*cos(THE_Psi_pend)+sin(THE_Phi_pend).*sin(THE_Psi_pend).*sin(THE_Theta_pend)).*(THE_Theta_D.*cos(THE_Psi)+THE_Phi_D.*cos(THE_Theta).*sin(THE_Psi))+THE_Theta_pend_D.*cos(THE_Psi_pend)-(THE_Psi_D-THE_Phi_D.*sin(THE_Theta)).*(cos(THE_Psi_pend).*sin(THE_Phi_pend)-cos(THE_Phi_pend).*sin(THE_Psi_pend).*sin(THE_Theta_pend))+THE_Phi_pend_D.*cos(THE_Theta_pend).*sin(THE_Psi_pend)-cos(THE_Theta_pend).*sin(THE_Psi_pend).*(THE_Theta_D.*sin(THE_Psi)-THE_Phi_D.*cos(THE_Psi).*cos(THE_Theta)))-m_pend.*(Lx_pend.^2./1.2e+1+Lz_pend.^2./1.2e+1).*((cos(THE_Phi_pend).*sin(THE_Psi_pend)-cos(THE_Psi_pend).*sin(THE_Phi_pend).*sin(THE_Theta_pend)).*(THE_Theta_D.*cos(THE_Psi)+THE_Phi_D.*cos(THE_Theta).*sin(THE_Psi))-(THE_Psi_D-THE_Phi_D.*sin(THE_Theta)).*(sin(THE_Phi_pend).*sin(THE_Psi_pend)+cos(THE_Phi_pend).*cos(THE_Psi_pend).*sin(THE_Theta_pend))+THE_Theta_pend_D.*sin(THE_Psi_pend)-THE_Phi_pend_D.*cos(THE_Psi_pend).*cos(THE_Theta_pend)+cos(THE_Psi_pend).*cos(THE_Theta_pend).*(THE_Theta_D.*sin(THE_Psi)-THE_Phi_D.*cos(THE_Psi).*cos(THE_Theta))).*(((cos(THE_Phi_pend).*cos(THE_Psi_pend)+sin(THE_Phi_pend).*sin(THE_Psi_pend).*sin(THE_Theta_pend)).*(THE_Theta_D.*cos(THE_Psi)+THE_Phi_D.*cos(THE_Theta).*sin(THE_Psi)))./2.0+(THE_Theta_pend_D.*cos(THE_Psi_pend))./2.0-((THE_Psi_D-THE_Phi_D.*sin(THE_Theta)).*(cos(THE_Psi_pend).*sin(THE_Phi_pend)-cos(THE_Phi_pend).*sin(THE_Psi_pend).*sin(THE_Theta_pend)))./2.0+(THE_Phi_pend_D.*cos(THE_Theta_pend).*sin(THE_Psi_pend))./2.0-(cos(THE_Theta_pend).*sin(THE_Psi_pend).*(THE_Theta_D.*sin(THE_Psi)-THE_Phi_D.*cos(THE_Psi).*cos(THE_Theta)))./2.0)-m_pend.*(Lx_pend.^2./1.2e+1+Lz_pend.^2./1.2e+1).*(((cos(THE_Phi_pend).*sin(THE_Psi_pend)-cos(THE_Psi_pend).*sin(THE_Phi_pend).*sin(THE_Theta_pend)).*(THE_Theta_D.*cos(THE_Psi)+THE_Phi_D.*cos(THE_Theta).*sin(THE_Psi)))./2.0-((THE_Psi_D-THE_Phi_D.*sin(THE_Theta)).*(sin(THE_Phi_pend).*sin(THE_Psi_pend)+cos(THE_Phi_pend).*cos(THE_Psi_pend).*sin(THE_Theta_pend)))./2.0+(THE_Theta_pend_D.*sin(THE_Psi_pend))./2.0-(THE_Phi_pend_D.*cos(THE_Psi_pend).*cos(THE_Theta_pend))./2.0+(cos(THE_Psi_pend).*cos(THE_Theta_pend).*(THE_Theta_D.*sin(THE_Psi)-THE_Phi_D.*cos(THE_Psi).*cos(THE_Theta)))./2.0).*((cos(THE_Phi_pend).*cos(THE_Psi_pend)+sin(THE_Phi_pend).*sin(THE_Psi_pend).*sin(THE_Theta_pend)).*(THE_Theta_D.*cos(THE_Psi)+THE_Phi_D.*cos(THE_Theta).*sin(THE_Psi))+THE_Theta_pend_D.*cos(THE_Psi_pend)-(THE_Psi_D-THE_Phi_D.*sin(THE_Theta)).*(cos(THE_Psi_pend).*sin(THE_Phi_pend)-cos(THE_Phi_pend).*sin(THE_Psi_pend).*sin(THE_Theta_pend))+THE_Phi_pend_D.*cos(THE_Theta_pend).*sin(THE_Psi_pend)-cos(THE_Theta_pend).*sin(THE_Psi_pend).*(THE_Theta_D.*sin(THE_Psi)-THE_Phi_D.*cos(THE_Psi).*cos(THE_Theta)))];
end
